simulink library "ammclib_bam_S32K3xx"  (R2016a)
settings: Solver=VariableStepAuto  SolverMode=SingleTasking  StartTime=0.0  StopTime=10.0  RelTol=1e-3
undefined symbols (not defined in the file or in its folder): a1, a2, ADCMaxError, autoCalcEn, b0, b1, b2, cfg, dgain, escale, f16A1, f16A2, f16ADCMaxError, f16B0, f16B1, f16B2, f16C1, f16CC1sc, f16CC1sc_D, f16CC1sc_Q, f16CC2sc, f16CC2sc_D, f16CC2sc_Q, f16DerivGain, f16EGain, f16FiltCoef, f16HystOff, f16HystOn, f16IGain, f16IntegGain, f16IntegGain_D, f16IntegGain_Q, f16IntegGainQ, f16Kd, f16KLs, f16Kq, f16KRs, f16Limit, f16LowerLimit, f16LowerLimit_D, f16LowerLimit_Q, f16LowerLimitQ, f16ModIndex, f16OutValOff, f16OutValOn, f16PropGain, f16PropGain_D, f16PropGain_Q, f16PropGainQ, f16RampDown, f16RampUp, f16UGain, f16UpperLimit, f16UpperLimit_D, f16UpperLimit_Q, f16UpperLimitQ, f16WIGain, f32A1, f32A2, f32ADCMaxError ... (+180)
(part 31 of 50)

== system ammclib_bam_S32K3xx/GFLIB/F16 ==
  GFLIB_Acos_F16 : Subsystem  TreatAsAtomicUnit=on  mask(GFLIB_Acos_F16){}
      mask help: Inverse cosine function in 16-bit fixed-point fractional implementation. Refer to the AMMCLIB User's Guide for further details.
      mask init: same as ammclib_bam_S32K3xx/GDFLIB/F16/GDFLIB_FilterFIR_F16
      settings: RTWSystemCode=Inline
      mask Help: web([fileparts(which('ammclib_bam_S32K3xx.slx')) '/../doc/S32K3XXMCLUG.pdf'], '-browser')
      mask Display: pos = get_param(gcb, 'Position');width = pos(3) - pos(1); height = pos(4) - pos(2);tX=width/2;tY=height - 8;color('black');text(tX,tY, 'GFLIB_Acos_F16', 'horizontalAlignment', 'center');
  GFLIB_Asin_F16 : Subsystem  TreatAsAtomicUnit=on  mask(GFLIB_Asin_F16){}
      mask help: Inverse sine function in 16-bit fixed-point fractional implementation. Refer to the AMMCLIB User's Guide for further details.
      mask init: same as ammclib_bam_S32K3xx/GDFLIB/F16/GDFLIB_FilterFIR_F16
      settings: RTWSystemCode=Inline
      mask Help: web([fileparts(which('ammclib_bam_S32K3xx.slx')) '/../doc/S32K3XXMCLUG.pdf'], '-browser')
      mask Display: pos = get_param(gcb, 'Position');width = pos(3) - pos(1); height = pos(4) - pos(2);tX=width/2;tY=height - 8;color('black');text(tX,tY, 'GFLIB_Asin_F16', 'horizontalAlignment', 'center');
  GFLIB_AtanYXShifted_F16 : Subsystem  TreatAsAtomicUnit=on  mask(GFLIB_AtanYXShifted_F16){}
      mask help: Shifted arctangent of two arguments Y/X in 16-bit fixed-point fractional implementation. Refer to the AMMCLIB User's Guide for further details.
      mask init: same as ammclib_bam_S32K3xx/GDFLIB/F16/GDFLIB_FilterFIR_F16
      settings: RTWSystemCode=Inline
      mask Help: web([fileparts(which('ammclib_bam_S32K3xx.slx')) '/../doc/S32K3XXMCLUG.pdf'], '-browser')
      mask Display: pos = get_param(gcb, 'Position');width = pos(3) - pos(1); height = pos(4) - pos(2);tX=width/2;tY=height - 8;color('black');text(tX,tY, 'GFLIB_AtanYXShifted_F16', 'horizontalAlignment', 'center');
  GFLIB_AtanYX_F16 : Subsystem  TreatAsAtomicUnit=on  mask(GFLIB_AtanYX_F16){}
      mask help: Arctangent of two arguments Y/X in 16-bit fixed-point fractional implementation. Refer to the AMMCLIB User's Guide for further details.
      mask init: same as ammclib_bam_S32K3xx/GDFLIB/F16/GDFLIB_FilterFIR_F16
      settings: RTWSystemCode=Inline
      mask Help: web([fileparts(which('ammclib_bam_S32K3xx.slx')) '/../doc/S32K3XXMCLUG.pdf'], '-browser')
      mask Display: pos = get_param(gcb, 'Position');width = pos(3) - pos(1); height = pos(4) - pos(2);tX=width/2;tY=height - 8;color('black');text(tX,tY, 'GFLIB_AtanYX_F16', 'horizontalAlignment', 'center');
  GFLIB_Atan_F16 : Subsystem  TreatAsAtomicUnit=on  mask(GFLIB_Atan_F16){}
      mask help: Inverse tangent function in 16-bit fixed-point fractional implementation. Refer to the AMMCLIB User's Guide for further details.
      mask init: same as ammclib_bam_S32K3xx/GDFLIB/F16/GDFLIB_FilterFIR_F16
      settings: RTWSystemCode=Inline
      mask Help: web([fileparts(which('ammclib_bam_S32K3xx.slx')) '/../doc/S32K3XXMCLUG.pdf'], '-browser')
      mask Display: pos = get_param(gcb, 'Position');width = pos(3) - pos(1); height = pos(4) - pos(2);tX=width/2;tY=height - 8;color('black');text(tX,tY, 'GFLIB_Atan_F16', 'horizontalAlignment', 'center');
  GFLIB_ControllerPIDpAW_F16 : Subsystem  StartFcn=|  TreatAsAtomicUnit=on  mask(GFLIB_ControllerPIDpAW_F16){showStates=Hide (faster execution), resetStatesEnable=Pre-set according to the first set of inputs after reset, SampleTime=-1, pgain=5, igain=0.5, dgain=0.01, filtCoef=10, lowerLimit=-10, upperLimit=9.99969482421875, inscale=10, outscale=10, autoCalcEn=on, f16PropGain=0, f16IntegGain=0, f16DerivGain=0, f16FiltCoef=0, s16PropGainShift=0, s16IntegGainShift=0, s16DerivGainShift=0, f16LowerLimit=0, f16UpperLimit=0, SampleTime_1=NaN}
      | ts=get_param(gcb,'CompiledSampleTime');
      | if iscell(ts)
      |   ts=ts{1};
      |   if iscell(ts)
      |     ts=ts{1};
      |   end
      | end
      | ts=ts(1);
      | set_param(gcb,'SampleTime_1',num2str(ts));
      | p=Simulink.Mask.get(gcb);
      | hintText=p.getDialogControl('timeHint');
      | SampleTime=Simulink.data.evalinGlobal(bdroot,get_param(gcb,'SampleTime'));
      | p=Simulink.Mask.get(gcb);
      | autoCalcEn=get_param(gcb,'autoCalcEn');
      | if strcmp(autoCalcEn,'on')
      |   if SampleTime==-1
      |     hintText.Prompt='Caution: Implementation parameters depend on inherited sample time. Make sure that the sample time of the block''s inputs corresponds to the sampling period in the target application.';
      |   else
      |     hintText.Prompt='Caution: Implementation parameters depend on the sample time. Make sure that the simulation time step corresponds to the sampling period in the target application.';
      |   end
      |   SampleTime=ts;
      |   f16PropGain_bkup=get_param(gcb,'f16PropGain');
      |   f16IntegGain_bkup=get_param(gcb,'f16IntegGain');
      |   f16DerivGain_bkup=get_param(gcb,'f16DerivGain');
      |   f16FiltCoef_bkup=get_param(gcb,'f16FiltCoef');
      |   s16PropGainShift_bkup=get_param(gcb,'s16PropGainShift');
      |   s16IntegGainShift_bkup=get_param(gcb,'s16IntegGainShift');
      |   s16DerivGainShift_bkup=get_param(gcb,'s16DerivGainShift');
      |   f16LowerLimit_bkup=get_param(gcb,'f16LowerLimit');
      |   f16UpperLimit_bkup=get_param(gcb,'f16UpperLimit');
      |   pgain=Simulink.data.evalinGlobal(bdroot,get_param(gcb,'pgain'));
      |   igain=Simulink.data.evalinGlobal(bdroot,get_param(gcb,'igain'));
      |   dgain=Simulink.data.evalinGlobal(bdroot,get_param(gcb,'dgain'));
      |   filtCoef=Simulink.data.evalinGlobal(bdroot,get_param(gcb,'filtCoef'));
      |   lowerLimit=Simulink.data.evalinGlobal(bdroot,get_param(gcb,'lowerLimit'));
      |   upperLimit=Simulink.data.evalinGlobal(bdroot,get_param(gcb,'upperLimit'));
      |   inscale=Simulink.data.evalinGlobal(bdroot,get_param(gcb,'inscale'));
      |   outscale=Simulink.data.evalinGlobal(bdroot,get_param(gcb,'outscale'));
      |   if (upperLimit<=lowerLimit)
      |     warning('UpperLimit should be greater than LowerLimit.');
      |   end
      |   if (inscale<=0)
      |     warning('E_max must be positive.');
      |   end
      |   if (outscale<=0)
      |     warning('U_max must be positive.');
      |   end
      |   kpf=pgain*inscale/outscale;
      |   s16PropGainShift=ceil(log2(abs(kpf)));
      |   if s16PropGainShift<-15
      |     s16PropGainShift=-15;
      |   end
      |   if s16PropGainShift>15
      |     s16PropGainShift=15;
      |     warning(['Parameter s16PropGainShift of ' gcb ' exceeds the fixed-point range.']);
      |   end
      |   f16PropGain=round(kpf*2^(-s16PropGainShift)*2^15);
      |   if f16PropGain>2^15-1
      |     f16PropGain=2^15-1;
      |     warning(['Parameter f16PropGain of ' gcb ' exceeds the fixed-point range.']);
      |   end
      |   if f16PropGain<-2^15
      |     f16PropGain=-2^15;
      |     warning(['Parameter f16PropGain of ' gcb ' exceeds the fixed-point range.']);
      |   end
      |   kif=igain*SampleTime*0.5*inscale/outscale;
      |   s16IntegGainShift=ceil(log2(abs(kif)));
      |   if s16IntegGainShift<-15
      |     s16IntegGainShift=-15;
      |   end
      |   if s16IntegGainShift>15
      |     s16IntegGainShift=15;
      |     warning(['Parameter s16IntegGainShift of ' gcb ' exceeds the fixed-point range.']);
      |   end
      |   f16IntegGain=round(kif*2^(-s16IntegGainShift)*2^15);
      |   if f16IntegGain>2^15-1
      |     f16IntegGain=2^15-1;
      |     warning(['Parameter f16IntegGain of ' gcb ' exceeds the fixed-point range.']);
      |   end
      |   if f16IntegGain<-2^15
      |     f16IntegGain=-2^15;
      |     warning(['Parameter f16IntegGain of ' gcb ' exceeds the fixed-point range.']);
      |   end
      |   upperLimitf=upperLimit/outscale;
      |   lowerLimitf=lowerLimit/outscale;
      |   f16UpperLimit=round(upperLimitf*2^15);
      |   if f16UpperLimit>2^15-1
      |     f16UpperLimit=2^15-1;
      |     warning(['Parameter f16UpperLimit of ' gcb ' exceeds the fixed-point range.']);
      |   end
      |   if f16UpperLimit<-2^15
      |     f16UpperLimit=-2^15;
      |     warning(['Parameter f16UpperLimit of ' gcb ' exceeds the fixed-point range.']);
      |   end
      |   f16LowerLimit=round(lowerLimitf*2^15);
      |   if f16LowerLimit>2^15-1
      |     f16LowerLimit=2^15-1;
      |     warning(['Parameter f16LowerLimit of ' gcb ' exceeds the fixed-point range.']);
      |   end
      |   if f16LowerLimit<-2^15
      |     f16LowerLimit=-2^15;
      |     warning(['Parameter f16LowerLimit of ' gcb ' exceeds the fixed-point range.']);
      |   end
      |   exparg=-SampleTime*filtCoef;
      |   expconst=exp(exparg);
      |   f16FiltCoef=round(expconst*2^15);
      |   if f16FiltCoef>2^15-1
      |     f16FiltCoef=2^15-1;
      |     warning(['Parameter f16FiltCoef of ' gcb ' exceeds the fixed-point range.']);
      |   end
      |   if f16FiltCoef<-2^15
      |     f16FiltCoef=-2^15;
      |     warning(['Parameter f16FiltCoef of ' gcb ' exceeds the fixed-point range.']);
      |   end
      |   kdf=dgain/SampleTime*(1 - expconst)*inscale/outscale;
      |   s16DerivGainShift=ceil(log2(abs(kpf)));
      |   if s16DerivGainShift<-15
      |     s16DerivGainShift=-15;
      |   end
      |   if s16DerivGainShift>15
      |     s16DerivGainShift=15;
      |     warning(['Parameter s16DerivGainShift of ' gcb ' exceeds the fixed-point range.']);
      |   end
      |   f16DerivGain=round(kpf*2^(-s16DerivGainShift)*2^15);
      |   if f16DerivGain>2^15-1
      |     f16DerivGain=2^15-1;
      |     warning(['Parameter f16DerivGain of ' gcb ' exceeds the fixed-point range.']);
      |   end
      |   if f16DerivGain<-2^15
      |     f16DerivGain=-2^15;
      |     warning(['Parameter f16DerivGain of ' gcb ' exceeds the fixed-point range.']);
      |   end
      |   if isnan(f16PropGain)
      |     if ~strcmp(f16PropGain_bkup,'0')
      |       set_param(gcb,'f16PropGain','0');
      |     end
      |   else
      |     tmps=num2str(f16PropGain);
      |     if ~strcmp(f16PropGain_bkup,tmps)
      |       set_param(gcb,'f16PropGain',tmps);
      |     end
      |   end
      |   if isnan(f16IntegGain)
      |     if ~strcmp(f16IntegGain_bkup,'0')
      |       set_param(gcb,'f16IntegGain','0');
      |     end
      |   else
      |     tmps=num2str(f16IntegGain);
      |     if ~strcmp(f16IntegGain_bkup,tmps)
      |       set_param(gcb,'f16IntegGain',tmps);
      |     end
      |   end
      |   if isnan(f16DerivGain)
      |     if ~strcmp(f16DerivGain_bkup,'0')
      |       set_param(gcb,'f16DerivGain','0');
      |     end
      |   else
      |     tmps=num2str(f16DerivGain);
      |     if ~strcmp(f16DerivGain_bkup,tmps)
      |       set_param(gcb,'f16DerivGain',tmps);
      |     end
      |   end
      |   if isnan(f16FiltCoef)
      |     if ~strcmp(f16FiltCoef_bkup,'0')
      |       set_param(gcb,'f16FiltCoef','0');
      |     end
      |   else
      |     tmps=num2str(f16FiltCoef);
      |     if ~strcmp(f16FiltCoef_bkup,tmps)
      |       set_param(gcb,'f16FiltCoef',tmps);
      |     end
      |   end
      |   if isnan(s16PropGainShift)
      |     if ~strcmp(s16PropGainShift_bkup,'0')
      |       set_param(gcb,'s16PropGainShift','0');
      |     end
      |   else
      |     tmps=num2str(s16PropGainShift);
      |     if ~strcmp(s16PropGainShift_bkup,tmps)
      |       set_param(gcb,'s16PropGainShift',tmps);
      |     end
      |   end
      |   if isnan(s16IntegGainShift)
      |     if ~strcmp(s16IntegGainShift_bkup,'0')
      |       set_param(gcb,'s16IntegGainShift','0');
      |     end
      |   else
      |     tmps=num2str(s16IntegGainShift);
      |     if ~strcmp(s16IntegGainShift_bkup,tmps)
      |       set_param(gcb,'s16IntegGainShift',tmps);
      |     end
      |   end
      |   if isnan(s16DerivGainShift)
      |     if ~strcmp(s16DerivGainShift_bkup,'0')
      |       set_param(gcb,'s16DerivGainShift','0');
      |     end
      |   else
      |     tmps=num2str(s16DerivGainShift);
      |     if ~strcmp(s16DerivGainShift_bkup,tmps)
      |       set_param(gcb,'s16DerivGainShift',tmps);
      |     end
      |   end
      |   if isnan(f16LowerLimit)
      |     if ~strcmp(f16LowerLimit_bkup,'0')
      |       set_param(gcb,'f16LowerLimit','0');
      |     end
      |   else
      |     tmps=num2str(f16LowerLimit);
      |     if ~strcmp(f16LowerLimit_bkup,tmps)
      |       set_param(gcb,'f16LowerLimit',tmps);
      |     end
      |   end
      |   if isnan(f16UpperLimit)
      |     if ~strcmp(f16UpperLimit_bkup,'0')
      |       set_param(gcb,'f16UpperLimit','0');
      |     end
      |   else
      |     tmps=num2str(f16UpperLimit);
      |     if ~strcmp(f16UpperLimit_bkup,tmps)
      |       set_param(gcb,'f16UpperLimit',tmps);
      |     end
      |   end
      | end
      mask prompts: showStates "Show internal states:"; resetStatesEnable "Internal state after reset:"; SampleTime "Sample time (-1 for inherited):"; pgain "Proportional gain (P):"; igain "Integral gain (I):"; dgain "Derivative gain (D):"; filtCoef "Derivative gain limit N (usually 3 to 20):"; lowerLimit "Controller lower limit:"; upperLimit "Controller upper limit:"; inscale "E_max (input scale):"; outscale "U_max (output scale):"; autoCalcEn "Calculate implementation parameters from physical parameters"; f16PropGain "f16PropGain (Proportional gain):"; f16IntegGain "f16IntegGain (Integral gain):"; f16DerivGain "f16DerivGain (Derivative gain):"; f16FiltCoef "f16FiltCoef (Derivative term filter coefficient):"; s16PropGainShift "s16PropGainShift (Proportional gain shift):"; s16IntegGainShift "s16IntegGainShift (Integral gain shift):"; s16DerivGainShift "s16DerivGainShift (Derivative gain shift):"; f16LowerLimit "f16LowerLimit (Lower limit of the controller):"; f16UpperLimit "f16UpperLimit (Upper limit of the controller):"; SampleTime_1 "Discrete sample time:"
      mask help: Parallel form of a discrete-time PID controller with anti-windup in 16-bit fixed-point fractional implementation. This block supports re-initialization of the internal state during simulation. If the block is reset, the controller's output will be aligned with the input f16ControllerPIDpAWOut_preset. Refer to the AMMCLIB User's Guide for further details.
      mask init:
      | ddName = get_param(bdroot,'DataDictionary');
      | if length(ddName)==0
      |   set_param(bdroot,'DataDictionary','ammclib_types.sldd');
      | else
      |   dd = Simulink.data.dictionary.open(ddName);
      |   data = getSection(dd,'Design Data');
      |   if ~exist(data,'SWLIBS_2Syst_F16')
      |     addDataSource(dd,'ammclib_types.sldd');
      |     saveChanges(dd);
      |   end
      | end
      | 
      | if showStates == 1
      |   % hidden state variables
      |   if strcmp(get_param([gcb '/f16PropGain'], 'BlockType'), 'Inport')
      |     posblk = get_param(gcb, 'Position');
      | 
      |     pos = get_param([gcb, '/f16PropGain'], 'Position');
      |     orient = get_param([gcb, '/f16PropGain'], 'Orientation');
      |     delete_block([gcb, '/f16PropGain']);
      |     add_block('built-in/Ground', [gcb, '/f16PropGain'], 'Position', pos, 'Orientation', orient);
      | 
      |     pos = get_param([gcb, '/f16IntegGain'], 'Position');
      |     orient = get_param([gcb, '/f16IntegGain'], 'Orientation');
      |     delete_block([gcb, '/f16IntegGain']);
      |     add_block('built-in/Ground', [gcb, '/f16IntegGain'], 'Position', pos, 'Orientation', orient);
      | 
      |     pos = get_param([gcb, '/f16DerivGain'], 'Position');
      |     orient = get_param([gcb, '/f16DerivGain'], 'Orientation');
      |     delete_block([gcb, '/f16DerivGain']);
      |     add_block('built-in/Ground', [gcb, '/f16DerivGain'], 'Position', pos, 'Orientation', orient);
      | 
      |     pos = get_param([gcb, '/f16FiltCoef'], 'Position');
      |     orient = get_param([gcb, '/f16FiltCoef'], 'Orientation');
      |     delete_block([gcb, '/f16FiltCoef']);
      |     add_block('built-in/Ground', [gcb, '/f16FiltCoef'], 'Position', pos, 'Orientation', orient);
      | 
      |     pos = get_param([gcb, '/s16PropGainShift'], 'Position');
      |     orient = get_param([gcb, '/s16PropGainShift'], 'Orientation');
      |     delete_block([gcb, '/s16PropGainShift']);
      |     add_block('built-in/Ground', [gcb, '/s16PropGainShift'], 'Position', pos, 'Orientation', orient);
      | 
      |     pos = get_param([gcb, '/s16IntegGainShift'], 'Position');
      |     orient = get_param([gcb, '/s16IntegGainShift'], 'Orientation');
      |     delete_block([gcb, '/s16IntegGainShift']);
      |     add_block('built-in/Ground', [gcb, '/s16IntegGainShift'], 'Position', pos, 'Orientation', orient);
      | 
      |     pos = get_param([gcb, '/s16DerivGainShift'], 'Position');
      |     orient = get_param([gcb, '/s16DerivGainShift'], 'Orientation');
      |     delete_block([gcb, '/s16DerivGainShift']);
      |     add_block('built-in/Ground', [gcb, '/s16DerivGainShift'], 'Position', pos, 'Orientation', orient);
      | 
      |     pos = get_param([gcb, '/f16LowerLimit'], 'Position');
      |     orient = get_param([gcb, '/f16LowerLimit'], 'Orientation');
      |     delete_block([gcb, '/f16LowerLimit']);
      |     add_block('built-in/Ground', [gcb, '/f16LowerLimit'], 'Position', pos, 'Orientation', orient);
      | 
      |     pos = get_param([gcb, '/f16UpperLimit'], 'Position');
      |     orient = get_param([gcb, '/f16UpperLimit'], 'Orientation');
      |     delete_block([gcb, '/f16UpperLimit']);
      |     add_block('built-in/Ground', [gcb, '/f16UpperLimit'], 'Position', pos, 'Orientation', orient);
      | 
      |     pos = get_param([gcb, '/f32IntegPartK_1'], 'Position');
      |     orient = get_param([gcb, '/f32IntegPartK_1'], 'Orientation');
      |     delete_block([gcb, '/f32IntegPartK_1']);
      |     add_block('built-in/Ground', [gcb, '/f32IntegPartK_1'], 'Position', pos, 'Orientation', orient);
      | 
      |     pos = get_param([gcb, '/f16DerivPartK_1'], 'Position');
      |     orient = get_param([gcb, '/f16DerivPartK_1'], 'Orientation');
      |     delete_block([gcb, '/f16DerivPartK_1']);
      |     add_block('built-in/Ground', [gcb, '/f16DerivPartK_1'], 'Position', pos, 'Orientation', orient);
      | 
      |     pos = get_param([gcb, '/f16InK_1'], 'Position');
      |     orient = get_param([gcb, '/f16InK_1'], 'Orientation');
      |     delete_block([gcb, '/f16InK_1']);
      |     add_block('built-in/Ground', [gcb, '/f16InK_1'], 'Position', pos, 'Orientation', orient);
      | 
      | 
      |     pmask=Simulink.Mask.get(gcb);
      |     pctrl=pmask.getParameter('SampleTime');
      |     pctrl.set('TypeOptions',{'f16InErr/SampleTime','f16ControllerPIDpAWOut_preset/SampleTime'});
      | 
      |     pos = get_param([gcb '/f32IntegPartK_1_Out'], 'Position');
      |     orient = get_param([gcb '/f32IntegPartK_1_Out'], 'Orientation');
      |     delete_block([gcb '/f32IntegPartK_1_Out']);
      |     add_block('built-in/Terminator', [gcb '/f32IntegPartK_1_Out'], 'Position', pos, 'Orientation', orient);
      | 
      |     pos = get_param([gcb '/f16DerivPartK_1_Out'], 'Position');
      |     orient = get_param([gcb '/f16DerivPartK_1_Out'], 'Orientation');
      |     delete_block([gcb '/f16DerivPartK_1_Out']);
      |     add_block('built-in/Terminator', [gcb '/f16DerivPartK_1_Out'], 'Position', pos, 'Orientation', orient);
      | 
      |     pos = get_param([gcb '/f16InK_1_Out'], 'Position');
      |     orient = get_param([gcb '/f16InK_1_Out'], 'Orientation');
      |     delete_block([gcb '/f16InK_1_Out']);
      |     add_block('built-in/Terminator', [gcb '/f16InK_1_Out'], 'Position', pos, 'Orientation', orient);
      | 
      |     set_param([gcb '/f16InErr'], 'Port', '1');
      |     set_param([gcb '/f16ControllerPIDpAWOut_preset'], 'Port', '2');
      | 
      |     tmpOutCnt=0;
      |     tmpOutCnt=tmpOutCnt+1;
      |     set_param([gcb '/f16Out'], 'Port', num2str(tmpOutCnt));
      |     tmpOutCnt=tmpOutCnt+1;
      |     set_param([gcb '/u16LimitFlag'], 'Port', num2str(tmpOutCnt));
      | 
      |     autoCalcEn=get_param(gcb,'autoCalcEn');
      |     if strcmp(autoCalcEn,'on')
      |       set_param(gcb,'MaskEnables',{'on','on','on','on','on','on','on','on','on','on','on','on','on','on','on','on','on','on','on','on','on','off'});
      |     else
      |       set_param(gcb,'MaskEnables',{'on','on','on','off','off','off','off','off','off','off','off','on','on','on','on','on','on','on','on','on','on','off'});
      |     end
      | 
      |     if (posblk(4) - posblk(2)) > 75
      |       height = 75;
      |       set_param(gcb,'Position',[posblk(1), posblk(2), posblk(3), posblk(2)+height])
      |     end
      |   end
      | else
      |   % shown state variables
      |   if strcmp(get_param([gcb '/f16PropGain'], 'BlockType'), 'Ground')
      |     posblk = get_param(gcb, 'Position');
      | 
      |     pos = get_param([gcb, '/f16PropGain'], 'Position');
      |     orient = get_param([gcb, '/f16PropGain'], 'Orientation');
      |     delete_block([gcb, '/f16PropGain']);
      |     add_block('built-in/Inport', [gcb, '/f16PropGain'], 'Position', pos, 'Orientation', orient, 'OutDataTypeStr', 'int16');
      | 
      |     pos = get_param([gcb, '/f16IntegGain'], 'Position');
      |     orient = get_param([gcb, '/f16IntegGain'], 'Orientation');
      |     delete_block([gcb, '/f16IntegGain']);
      |     add_block('built-in/Inport', [gcb, '/f16IntegGain'], 'Position', pos, 'Orientation', orient, 'OutDataTypeStr', 'int16');
      | 
      |     pos = get_param([gcb, '/f16DerivGain'], 'Position');
      |     orient = get_param([gcb, '/f16DerivGain'], 'Orientation');
      |     delete_block([gcb, '/f16DerivGain']);
      |     add_block('built-in/Inport', [gcb, '/f16DerivGain'], 'Position', pos, 'Orientation', orient, 'OutDataTypeStr', 'int16');
      | 
      |     pos = get_param([gcb, '/f16FiltCoef'], 'Position');
      |     orient = get_param([gcb, '/f16FiltCoef'], 'Orientation');
      |     delete_block([gcb, '/f16FiltCoef']);
      |     add_block('built-in/Inport', [gcb, '/f16FiltCoef'], 'Position', pos, 'Orientation', orient, 'OutDataTypeStr', 'int16');
      | 
      |     pos = get_param([gcb, '/s16PropGainShift'], 'Position');
      |     orient = get_param([gcb, '/s16PropGainShift'], 'Orientation');
      |     delete_block([gcb, '/s16PropGainShift']);
      |     add_block('built-in/Inport', [gcb, '/s16PropGainShift'], 'Position', pos, 'Orientation', orient, 'OutDataTypeStr', 'int16');
      | 
      |     pos = get_param([gcb, '/s16IntegGainShift'], 'Position');
      |     orient = get_param([gcb, '/s16IntegGainShift'], 'Orientation');
      |     delete_block([gcb, '/s16IntegGainShift']);
      |     add_block('built-in/Inport', [gcb, '/s16IntegGainShift'], 'Position', pos, 'Orientation', orient, 'OutDataTypeStr', 'int16');
      | 
      |     pos = get_param([gcb, '/s16DerivGainShift'], 'Position');
      |     orient = get_param([gcb, '/s16DerivGainShift'], 'Orientation');
      |     delete_block([gcb, '/s16DerivGainShift']);
      |     add_block('built-in/Inport', [gcb, '/s16DerivGainShift'], 'Position', pos, 'Orientation', orient, 'OutDataTypeStr', 'int16');
      | 
      |     pos = get_param([gcb, '/f16LowerLimit'], 'Position');
      |     orient = get_param([gcb, '/f16LowerLimit'], 'Orientation');
      |     delete_block([gcb, '/f16LowerLimit']);
      |     add_block('built-in/Inport', [gcb, '/f16LowerLimit'], 'Position', pos, 'Orientation', orient, 'OutDataTypeStr', 'int16');
      | 
      |     pos = get_param([gcb, '/f16UpperLimit'], 'Position');
      |     orient = get_param([gcb, '/f16UpperLimit'], 'Orientation');
      |     delete_block([gcb, '/f16UpperLimit']);
      |     add_block('built-in/Inport', [gcb, '/f16UpperLimit'], 'Position', pos, 'Orientation', orient, 'OutDataTypeStr', 'int16');
      | 
      |     pos = get_param([gcb, '/f32IntegPartK_1'], 'Position');
      |     orient = get_param([gcb, '/f32IntegPartK_1'], 'Orientation');
      |     delete_block([gcb, '/f32IntegPartK_1']);
      |     add_block('built-in/Inport', [gcb, '/f32IntegPartK_1'], 'Position', pos, 'Orientation', orient, 'OutDataTypeStr', 'int32');
      | 
      |     pos = get_param([gcb, '/f16DerivPartK_1'], 'Position');
      |     orient = get_param([gcb, '/f16DerivPartK_1'], 'Orientation');
      |     delete_block([gcb, '/f16DerivPartK_1']);
      |     add_block('built-in/Inport', [gcb, '/f16DerivPartK_1'], 'Position', pos, 'Orientation', orient, 'OutDataTypeStr', 'int16');
      | 
      |     pos = get_param([gcb, '/f16InK_1'], 'Position');
      |     orient = get_param([gcb, '/f16InK_1'], 'Orientation');
      |     delete_block([gcb, '/f16InK_1']);
      |     add_block('built-in/Inport', [gcb, '/f16InK_1'], 'Position', pos, 'Orientation', orient, 'OutDataTypeStr', 'int16');
      | 
      | 
      | 
      |     pos = get_param([gcb '/f32IntegPartK_1_Out'], 'Position');
      |     orient = get_param([gcb '/f32IntegPartK_1_Out'], 'Orientation');
      |     delete_block([gcb '/f32IntegPartK_1_Out']);
      |     add_block('built-in/Outport', [gcb '/f32IntegPartK_1_Out'], 'Position', pos, 'Orientation', orient);
      | 
      |     pos = get_param([gcb '/f16DerivPartK_1_Out'], 'Position');
      |     orient = get_param([gcb '/f16DerivPartK_1_Out'], 'Orientation');
      |     delete_block([gcb '/f16DerivPartK_1_Out']);
      |     add_block('built-in/Outport', [gcb '/f16DerivPartK_1_Out'], 'Position', pos, 'Orientation', orient);
      | 
      |     pos = get_param([gcb '/f16InK_1_Out'], 'Position');
      |     orient = get_param([gcb '/f16InK_1_Out'], 'Orientation');
      |     delete_block([gcb '/f16InK_1_Out']);
      |     add_block('built-in/Outport', [gcb '/f16InK_1_Out'], 'Position', pos, 'Orientation', orient);
      | 
      | 
      |     pmask=Simulink.Mask.get(gcb);
      |     pctrl=pmask.getParameter('SampleTime');
      |     pctrl.set('TypeOptions',{'f16InErr/SampleTime','f16ControllerPIDpAWOut_preset/SampleTime','f16PropGain/SampleTime','f16IntegGain/SampleTime','f16DerivGain/SampleTime','f16FiltCoef/SampleTime','s16PropGainShift/SampleTime','s16IntegGainShift/SampleTime','s16DerivGainShift/SampleTime','f16LowerLimit/SampleTime','f16UpperLimit/SampleTime','f32IntegPartK_1/SampleTime','f16DerivPartK_1/SampleTime','f16InK_1/SampleTime'});
      | 
      |     set_param([gcb '/f16InErr'], 'Port', '1');
      |     set_param([gcb '/f16ControllerPIDpAWOut_preset'], 'Port', '2');
      |     set_param([gcb '/f16PropGain'], 'Port', '3');
      |     set_param([gcb '/f16IntegGain'], 'Port', '4');
      |     set_param([gcb '/f16DerivGain'], 'Port', '5');
      |     set_param([gcb '/f16FiltCoef'], 'Port', '6');
      |     set_param([gcb '/s16PropGainShift'], 'Port', '7');
      |     set_param([gcb '/s16IntegGainShift'], 'Port', '8');
      |     set_param([gcb '/s16DerivGainShift'], 'Port', '9');
      |     set_param([gcb '/f16LowerLimit'], 'Port', '10');
      |     set_param([gcb '/f16UpperLimit'], 'Port', '11');
      |     set_param([gcb '/f32IntegPartK_1'], 'Port', '12');
      |     set_param([gcb '/f16DerivPartK_1'], 'Port', '13');
      |     set_param([gcb '/f16InK_1'], 'Port', '14');
      | 
      |     tmpOutCnt=0;
      |     tmpOutCnt=tmpOutCnt+1;
      |     set_param([gcb '/f16Out'], 'Port', num2str(tmpOutCnt));
      |     tmpOutCnt=tmpOutCnt+1;
      |     set_param([gcb '/u16LimitFlag'], 'Port', num2str(tmpOutCnt));
      |     tmpOutCnt=tmpOutCnt+1;
      |     set_param([gcb '/f32IntegPartK_1_Out'], 'Port', num2str(tmpOutCnt));
      |     tmpOutCnt=tmpOutCnt+1;
      |     set_param([gcb '/f16DerivPartK_1_Out'], 'Port', num2str(tmpOutCnt));
      |     tmpOutCnt=tmpOutCnt+1;
      |     set_param([gcb '/f16InK_1_Out'], 'Port', num2str(tmpOutCnt));
      | 
      |     set_param(gcb,'MaskEnables',{'on','on','on','off','off','off','off','off','off','off','off','off','off','off','off','off','off','off','off','off','off','off'});
      | 
      |     if (posblk(4) - posblk(2)) < 375
      |       height = 375;
      |       set_param(gcb,'Position',[posblk(1), posblk(2), posblk(3), posblk(2)+height])
      |     end
      |   end
      | end
      settings: RTWSystemCode=Inline
      mask Help: web([fileparts(which('ammclib_bam_S32K3xx.slx')) '/../doc/S32K3XXMCLUG.pdf'], '-browser')
      mask TypeOptions showStates: Hide (faster execution) | Show (allows debugging; connect feedback loops manually)
      mask Callback showStates:
      | maskStr=get_param(gcb,'showStates');
      | if strcmp(maskStr,'Hide (faster execution)')
      |   if strcmp(get_param([gcb '/f16PropGain'], 'BlockType'), 'Inport')
      |     autoCalcEn=get_param(gcb,'autoCalcEn');
      |     if strcmp(autoCalcEn,'on')
      |       set_param(gcb,'MaskEnables',{'on','on','on','on','on','on','on','on','on','on','on','on','on','on','on','on','on','on','on','on','on','off'});
      |     else
      |       set_param(gcb,'MaskEnables',{'on','on','on','off','off','off','off','off','off','off','off','on','on','on','on','on','on','on','on','on','on','off'});
      |     end
      |   end
      | else
      |   if strcmp(get_param([gcb '/f16PropGain'], 'BlockType'), 'Ground')
      |     set_param(gcb,'MaskEnables',{'on','on','on','off','off','off','off','off','off','off','off','off','off','off','off','off','off','off','off','off','off','off'});
      |   end
      | end
      mask TypeOptions resetStatesEnable: Pre-set according to the first set of inputs after reset | Clear to zero
      mask TypeOptions SampleTime: f16InErr/SampleTime | f16ControllerPIDpAWOut_preset/SampleTime
      mask Callback SampleTime:
      | p=Simulink.Mask.get(gcb);
      | hintText=p.getDialogControl('timeHint');
      | SampleTime=Simulink.data.evalinGlobal(bdroot,get_param(gcb,'SampleTime'));
      | SampleTime_1=str2double(get_param(gcb,'SampleTime_1'));
      | if (((SampleTime==-1) && (~contains(hintText.Prompt,'inherited'))) || ...
      |     ((SampleTime~=-1) && contains(hintText.Prompt,'inherited')) || ...
      |     ((SampleTime~=-1) && (SampleTime_1~=SampleTime)) || ...
      |     ((SampleTime_1~=-1) && contains(hintText.Prompt,'yet')))
      |   if ((SampleTime==-1) && (~contains(hintText.Prompt,'inherited')))
      |     set_param(gcb,'SampleTime_1',num2str(NaN));
      |     SampleTime_1=NaN;
      |   end
      |   if (SampleTime~=-1)
      |     set_param(gcb,'SampleTime_1',num2str(SampleTime));
      |     SampleTime_1=SampleTime;
      |   end
      |   autoCalcEn=get_param(gcb,'autoCalcEn');
      |   if strcmp(autoCalcEn,'on')
      |     p=Simulink.Mask.get(gcb);
      |     hintText=p.getDialogControl('timeHint');
      |     if SampleTime==-1
      |       SampleTime=SampleTime_1;
      |       if isnan(SampleTime)
      |         hintText.Prompt='Note: Implementation parameters cannot be calculated yet because the block''s inherited sample time is unknown. Simulink will update the sample time when you run the simulation.';
      |       else
      |         hintText.Prompt='Caution: Implementation parameters depend on inherited sample time. Make sure that the sample time of the block''s inputs corresponds to the sampling period in the target application.';
      |       end
      |     else
      |       hintText.Prompt='Caution: Implementation parameters depend on the sample time. Make sure that the simulation time step corresponds to the sampling period in the target application.';
      |     end
      |     f16PropGain_bkup=get_param(gcb,'f16PropGain');
      |     f16IntegGain_bkup=get_param(gcb,'f16IntegGain');
      |     f16DerivGain_bkup=get_param(gcb,'f16DerivGain');
      |     f16FiltCoef_bkup=get_param(gcb,'f16FiltCoef');
      |     s16PropGainShift_bkup=get_param(gcb,'s16PropGainShift');
      |     s16IntegGainShift_bkup=get_param(gcb,'s16IntegGainShift');
      |     s16DerivGainShift_bkup=get_param(gcb,'s16DerivGainShift');
      |     f16LowerLimit_bkup=get_param(gcb,'f16LowerLimit');
      |     f16UpperLimit_bkup=get_param(gcb,'f16UpperLimit');
      |     pgain=Simulink.data.evalinGlobal(bdroot,get_param(gcb,'pgain'));
      |     igain=Simulink.data.evalinGlobal(bdroot,get_param(gcb,'igain'));
      |     dgain=Simulink.data.evalinGlobal(bdroot,get_param(gcb,'dgain'));
      |     filtCoef=Simulink.data.evalinGlobal(bdroot,get_param(gcb,'filtCoef'));
      |     lowerLimit=Simulink.data.evalinGlobal(bdroot,get_param(gcb,'lowerLimit'));
      |     upperLimit=Simulink.data.evalinGlobal(bdroot,get_param(gcb,'upperLimit'));
      |     inscale=Simulink.data.evalinGlobal(bdroot,get_param(gcb,'inscale'));
      |     outscale=Simulink.data.evalinGlobal(bdroot,get_param(gcb,'outscale'));
      |     if (upperLimit<=lowerLimit)
      |       warning('UpperLimit should be greater than LowerLimit.');
      |     end
      |     if (inscale<=0)
      |       warning('E_max must be positive.');
      |     end
      |     if (outscale<=0)
      |       warning('U_max must be positive.');
      |     end
      |     kpf=pgain*inscale/outscale;
      |     s16PropGainShift=ceil(log2(abs(kpf)));
      |     if s16PropGainShift<-15
      |       s16PropGainShift=-15;
      |     end
      |     if s16PropGainShift>15
      |       s16PropGainShift=15;
      |       warning(['Parameter s16PropGainShift of ' gcb ' exceeds the fixed-point range.']);
      |     end
      |     f16PropGain=round(kpf*2^(-s16PropGainShift)*2^15);
      |     if f16PropGain>2^15-1
      |       f16PropGain=2^15-1;
      |       warning(['Parameter f16PropGain of ' gcb ' exceeds the fixed-point range.']);
      |     end
      |     if f16PropGain<-2^15
      |       f16PropGain=-2^15;
      |       warning(['Parameter f16PropGain of ' gcb ' exceeds the fixed-point range.']);
      |     end
      |     kif=igain*SampleTime*0.5*inscale/outscale;
      |     s16IntegGainShift=ceil(log2(abs(kif)));
      |     if s16IntegGainShift<-15
      |       s16IntegGainShift=-15;
      |     end
      |     if s16IntegGainShift>15
      |       s16IntegGainShift=15;
      |       warning(['Parameter s16IntegGainShift of ' gcb ' exceeds the fixed-point range.']);
      |     end
      |     f16IntegGain=round(kif*2^(-s16IntegGainShift)*2^15);
      |     if f16IntegGain>2^15-1
      |       f16IntegGain=2^15-1;
      |       warning(['Parameter f16IntegGain of ' gcb ' exceeds the fixed-point range.']);
      |     end
      |     if f16IntegGain<-2^15
      |       f16IntegGain=-2^15;
      |       warning(['Parameter f16IntegGain of ' gcb ' exceeds the fixed-point range.']);
      |     end
      |     upperLimitf=upperLimit/outscale;
      |     lowerLimitf=lowerLimit/outscale;
      |     f16UpperLimit=round(upperLimitf*2^15);
      |     if f16UpperLimit>2^15-1
      |       f16UpperLimit=2^15-1;
      |       warning(['Parameter f16UpperLimit of ' gcb ' exceeds the fixed-point range.']);
      |     end
      |     if f16UpperLimit<-2^15
      |       f16UpperLimit=-2^15;
      |       warning(['Parameter f16UpperLimit of ' gcb ' exceeds the fixed-point range.']);
      |     end
      |     f16LowerLimit=round(lowerLimitf*2^15);
      |     if f16LowerLimit>2^15-1
      |       f16LowerLimit=2^15-1;
      |       warning(['Parameter f16LowerLimit of ' gcb ' exceeds the fixed-point range.']);
      |     end
      |     if f16LowerLimit<-2^15
      |       f16LowerLimit=-2^15;
      |       warning(['Parameter f16LowerLimit of ' gcb ' exceeds the fixed-point range.']);
      |     end
      |     exparg=-SampleTime*filtCoef;
      |     expconst=exp(exparg);
      |     f16FiltCoef=round(expconst*2^15);
      |     if f16FiltCoef>2^15-1
      |       f16FiltCoef=2^15-1;
      |       warning(['Parameter f16FiltCoef of ' gcb ' exceeds the fixed-point range.']);
      |     end
      |     if f16FiltCoef<-2^15
      |       f16FiltCoef=-2^15;
      |       warning(['Parameter f16FiltCoef of ' gcb ' exceeds the fixed-point range.']);
      |     end
      |     kdf=dgain/SampleTime*(1 - expconst)*inscale/outscale;
      |     s16DerivGainShift=ceil(log2(abs(kpf)));
      |     if s16DerivGainShift<-15
      |       s16DerivGainShift=-15;
      |     end
      |     if s16DerivGainShift>15
      |       s16DerivGainShift=15;
      |       warning(['Parameter s16DerivGainShift of ' gcb ' exceeds the fixed-point range.']);
      |     end
      |     f16DerivGain=round(kpf*2^(-s16DerivGainShift)*2^15);
      |     if f16DerivGain>2^15-1
      |       f16DerivGain=2^15-1;
      |       warning(['Parameter f16DerivGain of ' gcb ' exceeds the fixed-point range.']);
      |     end
      |     if f16DerivGain<-2^15
      |       f16DerivGain=-2^15;
      |       warning(['Parameter f16DerivGain of ' gcb ' exceeds the fixed-point range.']);
      |     end
      |     if isnan(f16PropGain)
      |       if ~strcmp(f16PropGain_bkup,'0')
      |         set_param(gcb,'f16PropGain','0');
      |       end
      |     else
      |       tmps=num2str(f16PropGain);
      |       if ~strcmp(f16PropGain_bkup,tmps)
      |         set_param(gcb,'f16PropGain',tmps);
      |       end
      |     end
      |     if isnan(f16IntegGain)
      |       if ~strcmp(f16IntegGain_bkup,'0')
      |         set_param(gcb,'f16IntegGain','0');
      |       end
      |     else
      |       tmps=num2str(f16IntegGain);
      |       if ~strcmp(f16IntegGain_bkup,tmps)
      |         set_param(gcb,'f16IntegGain',tmps);
      |       end
      |     end
      |     if isnan(f16DerivGain)
      |       if ~strcmp(f16DerivGain_bkup,'0')
      |         set_param(gcb,'f16DerivGain','0');
      |       end
      |     else
      |       tmps=num2str(f16DerivGain);
      |       if ~strcmp(f16DerivGain_bkup,tmps)
      |         set_param(gcb,'f16DerivGain',tmps);
      |       end
      |     end
      |     if isnan(f16FiltCoef)
      |       if ~strcmp(f16FiltCoef_bkup,'0')
      |         set_param(gcb,'f16FiltCoef','0');
      |       end
      |     else
      |       tmps=num2str(f16FiltCoef);
      |       if ~strcmp(f16FiltCoef_bkup,tmps)
      |         set_param(gcb,'f16FiltCoef',tmps);
      |       end
      |     end
      |     if isnan(s16PropGainShift)
      |       if ~strcmp(s16PropGainShift_bkup,'0')
      |         set_param(gcb,'s16PropGainShift','0');
      |       end
      |     else
      |       tmps=num2str(s16PropGainShift);
      |       if ~strcmp(s16PropGainShift_bkup,tmps)
      |         set_param(gcb,'s16PropGainShift',tmps);
      |       end
      |     end
      |     if isnan(s16IntegGainShift)
      |       if ~strcmp(s16IntegGainShift_bkup,'0')
      |         set_param(gcb,'s16IntegGainShift','0');
      |       end
      |     else
      |       tmps=num2str(s16IntegGainShift);
      |       if ~strcmp(s16IntegGainShift_bkup,tmps)
      |         set_param(gcb,'s16IntegGainShift',tmps);
      |       end
      |     end
      |     if isnan(s16DerivGainShift)
      |       if ~strcmp(s16DerivGainShift_bkup,'0')
      |         set_param(gcb,'s16DerivGainShift','0');
      |       end
      |     else
      |       tmps=num2str(s16DerivGainShift);
      |       if ~strcmp(s16DerivGainShift_bkup,tmps)
      |         set_param(gcb,'s16DerivGainShift',tmps);
      |       end
      |     end
      |     if isnan(f16LowerLimit)
      |       if ~strcmp(f16LowerLimit_bkup,'0')
      |         set_param(gcb,'f16LowerLimit','0');
      |       end
      |     else
      |       tmps=num2str(f16LowerLimit);
      |       if ~strcmp(f16LowerLimit_bkup,tmps)
      |         set_param(gcb,'f16LowerLimit',tmps);
      |       end
      |     end
      |     if isnan(f16UpperLimit)
      |       if ~strcmp(f16UpperLimit_bkup,'0')
      |         set_param(gcb,'f16UpperLimit','0');
      |       end
      |     else
      |       tmps=num2str(f16UpperLimit);
      |       if ~strcmp(f16UpperLimit_bkup,tmps)
      |         set_param(gcb,'f16UpperLimit',tmps);
      |       end
      |     end
      |   end
      | end
      mask Callback pgain:
      | autoCalcEn=get_param(gcb,'autoCalcEn');
      | if strcmp(autoCalcEn,'on')
      |   SampleTime=Simulink.data.evalinGlobal(bdroot,get_param(gcb,'SampleTime'));
      |   if (SampleTime==-1)
      |     SampleTime=str2double(get_param(gcb,'SampleTime_1'));
      |   end
      |   f16PropGain_bkup=get_param(gcb,'f16PropGain');
      |   f16IntegGain_bkup=get_param(gcb,'f16IntegGain');
      |   f16DerivGain_bkup=get_param(gcb,'f16DerivGain');
      |   f16FiltCoef_bkup=get_param(gcb,'f16FiltCoef');
      |   s16PropGainShift_bkup=get_param(gcb,'s16PropGainShift');
      |   s16IntegGainShift_bkup=get_param(gcb,'s16IntegGainShift');
      |   s16DerivGainShift_bkup=get_param(gcb,'s16DerivGainShift');
      |   f16LowerLimit_bkup=get_param(gcb,'f16LowerLimit');
      |   f16UpperLimit_bkup=get_param(gcb,'f16UpperLimit');
      |   pgain=Simulink.data.evalinGlobal(bdroot,get_param(gcb,'pgain'));
      |   igain=Simulink.data.evalinGlobal(bdroot,get_param(gcb,'igain'));
      |   dgain=Simulink.data.evalinGlobal(bdroot,get_param(gcb,'dgain'));
      |   filtCoef=Simulink.data.evalinGlobal(bdroot,get_param(gcb,'filtCoef'));
      |   lowerLimit=Simulink.data.evalinGlobal(bdroot,get_param(gcb,'lowerLimit'));
      |   upperLimit=Simulink.data.evalinGlobal(bdroot,get_param(gcb,'upperLimit'));
      |   inscale=Simulink.data.evalinGlobal(bdroot,get_param(gcb,'inscale'));
      |   outscale=Simulink.data.evalinGlobal(bdroot,get_param(gcb,'outscale'));
      |   if (upperLimit<=lowerLimit)
      |     warning('UpperLimit should be greater than LowerLimit.');
      |   end
      |   if (inscale<=0)
      |     warning('E_max must be positive.');
      |   end
      |   if (outscale<=0)
      |     warning('U_max must be positive.');
      |   end
      |   kpf=pgain*inscale/outscale;
      |   s16PropGainShift=ceil(log2(abs(kpf)));
      |   if s16PropGainShift<-15
      |     s16PropGainShift=-15;
      |   end
      |   if s16PropGainShift>15
      |     s16PropGainShift=15;
      |     warning(['Parameter s16PropGainShift of ' gcb ' exceeds the fixed-point range.']);
      |   end
      |   f16PropGain=round(kpf*2^(-s16PropGainShift)*2^15);
      |   if f16PropGain>2^15-1
      |     f16PropGain=2^15-1;
      |     warning(['Parameter f16PropGain of ' gcb ' exceeds the fixed-point range.']);
      |   end
      |   if f16PropGain<-2^15
      |     f16PropGain=-2^15;
      |     warning(['Parameter f16PropGain of ' gcb ' exceeds the fixed-point range.']);
      |   end
      |   kif=igain*SampleTime*0.5*inscale/outscale;
      |   s16IntegGainShift=ceil(log2(abs(kif)));
      |   if s16IntegGainShift<-15
      |     s16IntegGainShift=-15;
      |   end
      |   if s16IntegGainShift>15
      |     s16IntegGainShift=15;
      |     warning(['Parameter s16IntegGainShift of ' gcb ' exceeds the fixed-point range.']);
      |   end
      |   f16IntegGain=round(kif*2^(-s16IntegGainShift)*2^15);
      |   if f16IntegGain>2^15-1
      |     f16IntegGain=2^15-1;
      |     warning(['Parameter f16IntegGain of ' gcb ' exceeds the fixed-point range.']);
      |   end
      |   if f16IntegGain<-2^15
      |     f16IntegGain=-2^15;
      |     warning(['Parameter f16IntegGain of ' gcb ' exceeds the fixed-point range.']);
      |   end
      |   upperLimitf=upperLimit/outscale;
      |   lowerLimitf=lowerLimit/outscale;
      |   f16UpperLimit=round(upperLimitf*2^15);
      |   if f16UpperLimit>2^15-1
      |     f16UpperLimit=2^15-1;
      |     warning(['Parameter f16UpperLimit of ' gcb ' exceeds the fixed-point range.']);
      |   end
      |   if f16UpperLimit<-2^15
      |     f16UpperLimit=-2^15;
      |     warning(['Parameter f16UpperLimit of ' gcb ' exceeds the fixed-point range.']);
      |   end
      |   f16LowerLimit=round(lowerLimitf*2^15);
      |   if f16LowerLimit>2^15-1
      |     f16LowerLimit=2^15-1;
      |     warning(['Parameter f16LowerLimit of ' gcb ' exceeds the fixed-point range.']);
      |   end
      |   if f16LowerLimit<-2^15
      |     f16LowerLimit=-2^15;
      |     warning(['Parameter f16LowerLimit of ' gcb ' exceeds the fixed-point range.']);
      |   end
      |   exparg=-SampleTime*filtCoef;
      |   expconst=exp(exparg);
      |   f16FiltCoef=round(expconst*2^15);
      |   if f16FiltCoef>2^15-1
      |     f16FiltCoef=2^15-1;
      |     warning(['Parameter f16FiltCoef of ' gcb ' exceeds the fixed-point range.']);
      |   end
      |   if f16FiltCoef<-2^15
      |     f16FiltCoef=-2^15;
      |     warning(['Parameter f16FiltCoef of ' gcb ' exceeds the fixed-point range.']);
      |   end
      |   kdf=dgain/SampleTime*(1 - expconst)*inscale/outscale;
      |   s16DerivGainShift=ceil(log2(abs(kpf)));
      |   if s16DerivGainShift<-15
      |     s16DerivGainShift=-15;
      |   end
      |   if s16DerivGainShift>15
      |     s16DerivGainShift=15;
      |     warning(['Parameter s16DerivGainShift of ' gcb ' exceeds the fixed-point range.']);
      |   end
      |   f16DerivGain=round(kpf*2^(-s16DerivGainShift)*2^15);
      |   if f16DerivGain>2^15-1
      |     f16DerivGain=2^15-1;
      |     warning(['Parameter f16DerivGain of ' gcb ' exceeds the fixed-point range.']);
      |   end
      |   if f16DerivGain<-2^15
      |     f16DerivGain=-2^15;
      |     warning(['Parameter f16DerivGain of ' gcb ' exceeds the fixed-point range.']);
      |   end
      |   if isnan(f16PropGain)
      |     if ~strcmp(f16PropGain_bkup,'0')
      |       set_param(gcb,'f16PropGain','0');
      |     end
      |   else
      |     tmps=num2str(f16PropGain);
      |     if ~strcmp(f16PropGain_bkup,tmps)
      |       set_param(gcb,'f16PropGain',tmps);
      |     end
      |   end
      |   if isnan(f16IntegGain)
      |     if ~strcmp(f16IntegGain_bkup,'0')
      |       set_param(gcb,'f16IntegGain','0');
      |     end
      |   else
      |     tmps=num2str(f16IntegGain);
      |     if ~strcmp(f16IntegGain_bkup,tmps)
      |       set_param(gcb,'f16IntegGain',tmps);
      |     end
      |   end
      |   if isnan(f16DerivGain)
      |     if ~strcmp(f16DerivGain_bkup,'0')
      |       set_param(gcb,'f16DerivGain','0');
      |     end
      |   else
      |     tmps=num2str(f16DerivGain);
      |     if ~strcmp(f16DerivGain_bkup,tmps)
      |       set_param(gcb,'f16DerivGain',tmps);
      |     end
      |   end
      |   if isnan(f16FiltCoef)
      |     if ~strcmp(f16FiltCoef_bkup,'0')
      |       set_param(gcb,'f16FiltCoef','0');
      |     end
      |   else
      |     tmps=num2str(f16FiltCoef);
      |     if ~strcmp(f16FiltCoef_bkup,tmps)
      |       set_param(gcb,'f16FiltCoef',tmps);
      |     end
      |   end
      |   if isnan(s16PropGainShift)
      |     if ~strcmp(s16PropGainShift_bkup,'0')
      |       set_param(gcb,'s16PropGainShift','0');
      |     end
      |   else
      |     tmps=num2str(s16PropGainShift);
      |     if ~strcmp(s16PropGainShift_bkup,tmps)
      |       set_param(gcb,'s16PropGainShift',tmps);
      |     end
      |   end
      |   if isnan(s16IntegGainShift)
      |     if ~strcmp(s16IntegGainShift_bkup,'0')
      |       set_param(gcb,'s16IntegGainShift','0');
      |     end
      |   else
      |     tmps=num2str(s16IntegGainShift);
      |     if ~strcmp(s16IntegGainShift_bkup,tmps)
      |       set_param(gcb,'s16IntegGainShift',tmps);
      |     end
      |   end
      |   if isnan(s16DerivGainShift)
      |     if ~strcmp(s16DerivGainShift_bkup,'0')
      |       set_param(gcb,'s16DerivGainShift','0');
      |     end
      |   else
      |     tmps=num2str(s16DerivGainShift);
      |     if ~strcmp(s16DerivGainShift_bkup,tmps)
      |       set_param(gcb,'s16DerivGainShift',tmps);
      |     end
      |   end
      |   if isnan(f16LowerLimit)
      |     if ~strcmp(f16LowerLimit_bkup,'0')
      |       set_param(gcb,'f16LowerLimit','0');
      |     end
      |   else
      |     tmps=num2str(f16LowerLimit);
      |     if ~strcmp(f16LowerLimit_bkup,tmps)
      |       set_param(gcb,'f16LowerLimit',tmps);
      |     end
      |   end
      |   if isnan(f16UpperLimit)
      |     if ~strcmp(f16UpperLimit_bkup,'0')
      |       set_param(gcb,'f16UpperLimit','0');
      |     end
      |   else
      |     tmps=num2str(f16UpperLimit);
      |     if ~strcmp(f16UpperLimit_bkup,tmps)
      |       set_param(gcb,'f16UpperLimit',tmps);
      |     end
      |   end
      | end
      mask Callback igain:
      | autoCalcEn=get_param(gcb,'autoCalcEn');
      | if strcmp(autoCalcEn,'on')
      |   SampleTime=Simulink.data.evalinGlobal(bdroot,get_param(gcb,'SampleTime'));
      |   if (SampleTime==-1)
      |     SampleTime=str2double(get_param(gcb,'SampleTime_1'));
      |   end
      |   f16PropGain_bkup=get_param(gcb,'f16PropGain');
      |   f16IntegGain_bkup=get_param(gcb,'f16IntegGain');
      |   f16DerivGain_bkup=get_param(gcb,'f16DerivGain');
      |   f16FiltCoef_bkup=get_param(gcb,'f16FiltCoef');
      |   s16PropGainShift_bkup=get_param(gcb,'s16PropGainShift');
      |   s16IntegGainShift_bkup=get_param(gcb,'s16IntegGainShift');
      |   s16DerivGainShift_bkup=get_param(gcb,'s16DerivGainShift');
      |   f16LowerLimit_bkup=get_param(gcb,'f16LowerLimit');
      |   f16UpperLimit_bkup=get_param(gcb,'f16UpperLimit');
      |   pgain=Simulink.data.evalinGlobal(bdroot,get_param(gcb,'pgain'));
      |   igain=Simulink.data.evalinGlobal(bdroot,get_param(gcb,'igain'));
      |   dgain=Simulink.data.evalinGlobal(bdroot,get_param(gcb,'dgain'));
      |   filtCoef=Simulink.data.evalinGlobal(bdroot,get_param(gcb,'filtCoef'));
      |   lowerLimit=Simulink.data.evalinGlobal(bdroot,get_param(gcb,'lowerLimit'));
      |   upperLimit=Simulink.data.evalinGlobal(bdroot,get_param(gcb,'upperLimit'));
      |   inscale=Simulink.data.evalinGlobal(bdroot,get_param(gcb,'inscale'));
      |   outscale=Simulink.data.evalinGlobal(bdroot,get_param(gcb,'outscale'));
      |   if (upperLimit<=lowerLimit)
      |     warning('UpperLimit should be greater than LowerLimit.');
      |   end
      |   if (inscale<=0)
      |     warning('E_max must be positive.');
      |   end
      |   if (outscale<=0)
      |     warning('U_max must be positive.');
      |   end
      |   kpf=pgain*inscale/outscale;
      |   s16PropGainShift=ceil(log2(abs(kpf)));
      |   if s16PropGainShift<-15
      |     s16PropGainShift=-15;
      |   end
      |   if s16PropGainShift>15
      |     s16PropGainShift=15;
      |     warning(['Parameter s16PropGainShift of ' gcb ' exceeds the fixed-point range.']);
      |   end
      |   f16PropGain=round(kpf*2^(-s16PropGainShift)*2^15);
      |   if f16PropGain>2^15-1
      |     f16PropGain=2^15-1;
      |     warning(['Parameter f16PropGain of ' gcb ' exceeds the fixed-point range.']);
      |   end
      |   if f16PropGain<-2^15
      |     f16PropGain=-2^15;
      |     warning(['Parameter f16PropGain of ' gcb ' exceeds the fixed-point range.']);
      |   end
      |   kif=igain*SampleTime*0.5*inscale/outscale;
      |   s16IntegGainShift=ceil(log2(abs(kif)));
      |   if s16IntegGainShift<-15
      |     s16IntegGainShift=-15;
      |   end
      |   if s16IntegGainShift>15
      |     s16IntegGainShift=15;
      |     warning(['Parameter s16IntegGainShift of ' gcb ' exceeds the fixed-point range.']);
      |   end
      |   f16IntegGain=round(kif*2^(-s16IntegGainShift)*2^15);
      |   if f16IntegGain>2^15-1
      |     f16IntegGain=2^15-1;
      |     warning(['Parameter f16IntegGain of ' gcb ' exceeds the fixed-point range.']);
      |   end
      |   if f16IntegGain<-2^15
      |     f16IntegGain=-2^15;
      |     warning(['Parameter f16IntegGain of ' gcb ' exceeds the fixed-point range.']);
      |   end
      |   upperLimitf=upperLimit/outscale;
      |   lowerLimitf=lowerLimit/outscale;
      |   f16UpperLimit=round(upperLimitf*2^15);
      |   if f16UpperLimit>2^15-1
      |     f16UpperLimit=2^15-1;
      |     warning(['Parameter f16UpperLimit of ' gcb ' exceeds the fixed-point range.']);
      |   end
      |   if f16UpperLimit<-2^15
      |     f16UpperLimit=-2^15;
      |     warning(['Parameter f16UpperLimit of ' gcb ' exceeds the fixed-point range.']);
      |   end
      |   f16LowerLimit=round(lowerLimitf*2^15);
      |   if f16LowerLimit>2^15-1
      |     f16LowerLimit=2^15-1;
      |     warning(['Parameter f16LowerLimit of ' gcb ' exceeds the fixed-point range.']);
      |   end
      |   if f16LowerLimit<-2^15
      |     f16LowerLimit=-2^15;
      |     warning(['Parameter f16LowerLimit of ' gcb ' exceeds the fixed-point range.']);
      |   end
      |   exparg=-SampleTime*filtCoef;
      |   expconst=exp(exparg);
      |   f16FiltCoef=round(expconst*2^15);
      |   if f16FiltCoef>2^15-1
      |     f16FiltCoef=2^15-1;
      |     warning(['Parameter f16FiltCoef of ' gcb ' exceeds the fixed-point range.']);
      |   end
      |   if f16FiltCoef<-2^15
      |     f16FiltCoef=-2^15;
      |     warning(['Parameter f16FiltCoef of ' gcb ' exceeds the fixed-point range.']);
      |   end
      |   kdf=dgain/SampleTime*(1 - expconst)*inscale/outscale;
      |   s16DerivGainShift=ceil(log2(abs(kpf)));
      |   if s16DerivGainShift<-15
      |     s16DerivGainShift=-15;
      |   end
      |   if s16DerivGainShift>15
      |     s16DerivGainShift=15;
      |     warning(['Parameter s16DerivGainShift of ' gcb ' exceeds the fixed-point range.']);
      |   end
      |   f16DerivGain=round(kpf*2^(-s16DerivGainShift)*2^15);
      |   if f16DerivGain>2^15-1
      |     f16DerivGain=2^15-1;
      |     warning(['Parameter f16DerivGain of ' gcb ' exceeds the fixed-point range.']);
      |   end
      |   if f16DerivGain<-2^15
      |     f16DerivGain=-2^15;
      |     warning(['Parameter f16DerivGain of ' gcb ' exceeds the fixed-point range.']);
      |   end
      |   if isnan(f16PropGain)
      |     if ~strcmp(f16PropGain_bkup,'0')
      |       set_param(gcb,'f16PropGain','0');
      |     end
      |   else
      |     tmps=num2str(f16PropGain);
      |     if ~strcmp(f16PropGain_bkup,tmps)
      |       set_param(gcb,'f16PropGain',tmps);
      |     end
      |   end
      |   if isnan(f16IntegGain)
      |     if ~strcmp(f16IntegGain_bkup,'0')
      |       set_param(gcb,'f16IntegGain','0');
      |     end
      |   else
      |     tmps=num2str(f16IntegGain);
      |     if ~strcmp(f16IntegGain_bkup,tmps)
      |       set_param(gcb,'f16IntegGain',tmps);
      |     end
      |   end
      |   if isnan(f16DerivGain)
      |     if ~strcmp(f16DerivGain_bkup,'0')
      |       set_param(gcb,'f16DerivGain','0');
      |     end
      |   else
      |     tmps=num2str(f16DerivGain);
      |     if ~strcmp(f16DerivGain_bkup,tmps)
      |       set_param(gcb,'f16DerivGain',tmps);
      |     end
      |   end
      |   if isnan(f16FiltCoef)
      |     if ~strcmp(f16FiltCoef_bkup,'0')
      |       set_param(gcb,'f16FiltCoef','0');
      |     end
      |   else
      |     tmps=num2str(f16FiltCoef);
      |     if ~strcmp(f16FiltCoef_bkup,tmps)
      |       set_param(gcb,'f16FiltCoef',tmps);
      |     end
      |   end
      |   if isnan(s16PropGainShift)
      |     if ~strcmp(s16PropGainShift_bkup,'0')
      |       set_param(gcb,'s16PropGainShift','0');
      |     end
      |   else
      |     tmps=num2str(s16PropGainShift);
      |     if ~strcmp(s16PropGainShift_bkup,tmps)
      |       set_param(gcb,'s16PropGainShift',tmps);
      |     end
      |   end
      |   if isnan(s16IntegGainShift)
      |     if ~strcmp(s16IntegGainShift_bkup,'0')
      |       set_param(gcb,'s16IntegGainShift','0');
      |     end
      |   else
      |     tmps=num2str(s16IntegGainShift);
      |     if ~strcmp(s16IntegGainShift_bkup,tmps)
      |       set_param(gcb,'s16IntegGainShift',tmps);
      |     end
      |   end
      |   if isnan(s16DerivGainShift)
      |     if ~strcmp(s16DerivGainShift_bkup,'0')
      |       set_param(gcb,'s16DerivGainShift','0');
      |     end
      |   else
      |     tmps=num2str(s16DerivGainShift);
      |     if ~strcmp(s16DerivGainShift_bkup,tmps)
      |       set_param(gcb,'s16DerivGainShift',tmps);
      |     end
      |   end
      |   if isnan(f16LowerLimit)
      |     if ~strcmp(f16LowerLimit_bkup,'0')
      |       set_param(gcb,'f16LowerLimit','0');
      |     end
      |   else
      |     tmps=num2str(f16LowerLimit);
      |     if ~strcmp(f16LowerLimit_bkup,tmps)
      |       set_param(gcb,'f16LowerLimit',tmps);
      |     end
      |   end
      |   if isnan(f16UpperLimit)
      |     if ~strcmp(f16UpperLimit_bkup,'0')
      |       set_param(gcb,'f16UpperLimit','0');
      |     end
      |   else
      |     tmps=num2str(f16UpperLimit);
      |     if ~strcmp(f16UpperLimit_bkup,tmps)
      |       set_param(gcb,'f16UpperLimit',tmps);
      |     end
      |   end
      | end
      mask Callback dgain:
      | autoCalcEn=get_param(gcb,'autoCalcEn');
      | if strcmp(autoCalcEn,'on')
      |   SampleTime=Simulink.data.evalinGlobal(bdroot,get_param(gcb,'SampleTime'));
      |   if (SampleTime==-1)
      |     SampleTime=str2double(get_param(gcb,'SampleTime_1'));
      |   end
      |   f16PropGain_bkup=get_param(gcb,'f16PropGain');
      |   f16IntegGain_bkup=get_param(gcb,'f16IntegGain');
      |   f16DerivGain_bkup=get_param(gcb,'f16DerivGain');
      |   f16FiltCoef_bkup=get_param(gcb,'f16FiltCoef');
      |   s16PropGainShift_bkup=get_param(gcb,'s16PropGainShift');
      |   s16IntegGainShift_bkup=get_param(gcb,'s16IntegGainShift');
      |   s16DerivGainShift_bkup=get_param(gcb,'s16DerivGainShift');
      |   f16LowerLimit_bkup=get_param(gcb,'f16LowerLimit');
      |   f16UpperLimit_bkup=get_param(gcb,'f16UpperLimit');
      |   pgain=Simulink.data.evalinGlobal(bdroot,get_param(gcb,'pgain'));
      |   igain=Simulink.data.evalinGlobal(bdroot,get_param(gcb,'igain'));
      |   dgain=Simulink.data.evalinGlobal(bdroot,get_param(gcb,'dgain'));
      |   filtCoef=Simulink.data.evalinGlobal(bdroot,get_param(gcb,'filtCoef'));
      |   lowerLimit=Simulink.data.evalinGlobal(bdroot,get_param(gcb,'lowerLimit'));
      |   upperLimit=Simulink.data.evalinGlobal(bdroot,get_param(gcb,'upperLimit'));
      |   inscale=Simulink.data.evalinGlobal(bdroot,get_param(gcb,'inscale'));
      |   outscale=Simulink.data.evalinGlobal(bdroot,get_param(gcb,'outscale'));
      |   if (upperLimit<=lowerLimit)
      |     warning('UpperLimit should be greater than LowerLimit.');
      |   end
      |   if (inscale<=0)
      |     warning('E_max must be positive.');
      |   end
      |   if (outscale<=0)
      |     warning('U_max must be positive.');
      |   end
      |   kpf=pgain*inscale/outscale;
      |   s16PropGainShift=ceil(log2(abs(kpf)));
      |   if s16PropGainShift<-15
      |     s16PropGainShift=-15;
      |   end
      |   if s16PropGainShift>15
      |     s16PropGainShift=15;
      |     warning(['Parameter s16PropGainShift of ' gcb ' exceeds the fixed-point range.']);
      |   end
      |   f16PropGain=round(kpf*2^(-s16PropGainShift)*2^15);
      |   if f16PropGain>2^15-1
      |     f16PropGain=2^15-1;
      |     warning(['Parameter f16PropGain of ' gcb ' exceeds the fixed-point range.']);
      |   end
      |   if f16PropGain<-2^15
      |     f16PropGain=-2^15;
      |     warning(['Parameter f16PropGain of ' gcb ' exceeds the fixed-point range.']);
      |   end
      |   kif=igain*SampleTime*0.5*inscale/outscale;
      |   s16IntegGainShift=ceil(log2(abs(kif)));
      |   if s16IntegGainShift<-15
      |     s16IntegGainShift=-15;
      |   end
      |   if s16IntegGainShift>15
      |     s16IntegGainShift=15;
      |     warning(['Parameter s16IntegGainShift of ' gcb ' exceeds the fixed-point range.']);
      |   end
      |   f16IntegGain=round(kif*2^(-s16IntegGainShift)*2^15);
      |   if f16IntegGain>2^15-1
      |     f16IntegGain=2^15-1;
      |     warning(['Parameter f16IntegGain of ' gcb ' exceeds the fixed-point range.']);
      |   end
      |   if f16IntegGain<-2^15
      |     f16IntegGain=-2^15;
      |     warning(['Parameter f16IntegGain of ' gcb ' exceeds the fixed-point range.']);
      |   end
      |   upperLimitf=upperLimit/outscale;
      |   lowerLimitf=lowerLimit/outscale;
      |   f16UpperLimit=round(upperLimitf*2^15);
      |   if f16UpperLimit>2^15-1
      |     f16UpperLimit=2^15-1;
      |     warning(['Parameter f16UpperLimit of ' gcb ' exceeds the fixed-point range.']);
      |   end
      |   if f16UpperLimit<-2^15
      |     f16UpperLimit=-2^15;
      |     warning(['Parameter f16UpperLimit of ' gcb ' exceeds the fixed-point range.']);
      |   end
      |   f16LowerLimit=round(lowerLimitf*2^15);
      |   if f16LowerLimit>2^15-1
      |     f16LowerLimit=2^15-1;
      |     warning(['Parameter f16LowerLimit of ' gcb ' exceeds the fixed-point range.']);
      |   end
      |   if f16LowerLimit<-2^15
      |     f16LowerLimit=-2^15;
      |     warning(['Parameter f16LowerLimit of ' gcb ' exceeds the fixed-point range.']);
      |   end
      |   exparg=-SampleTime*filtCoef;
      |   expconst=exp(exparg);
      |   f16FiltCoef=round(expconst*2^15);
      |   if f16FiltCoef>2^15-1
      |     f16FiltCoef=2^15-1;
      |     warning(['Parameter f16FiltCoef of ' gcb ' exceeds the fixed-point range.']);
      |   end
      |   if f16FiltCoef<-2^15
      |     f16FiltCoef=-2^15;
      |     warning(['Parameter f16FiltCoef of ' gcb ' exceeds the fixed-point range.']);
      |   end
      |   kdf=dgain/SampleTime*(1 - expconst)*inscale/outscale;
      |   s16DerivGainShift=ceil(log2(abs(kpf)));
      |   if s16DerivGainShift<-15
      |     s16DerivGainShift=-15;
      |   end
      |   if s16DerivGainShift>15
      |     s16DerivGainShift=15;
      |     warning(['Parameter s16DerivGainShift of ' gcb ' exceeds the fixed-point range.']);
      |   end
      |   f16DerivGain=round(kpf*2^(-s16DerivGainShift)*2^15);
      |   if f16DerivGain>2^15-1
      |     f16DerivGain=2^15-1;
      |     warning(['Parameter f16DerivGain of ' gcb ' exceeds the fixed-point range.']);
      |   end
      |   if f16DerivGain<-2^15
      |     f16DerivGain=-2^15;
      |     warning(['Parameter f16DerivGain of ' gcb ' exceeds the fixed-point range.']);
      |   end
      |   if isnan(f16PropGain)
      |     if ~strcmp(f16PropGain_bkup,'0')
      |       set_param(gcb,'f16PropGain','0');
      |     end
      |   else
      |     tmps=num2str(f16PropGain);
      |     if ~strcmp(f16PropGain_bkup,tmps)
      |       set_param(gcb,'f16PropGain',tmps);
      |     end
      |   end
      |   if isnan(f16IntegGain)
      |     if ~strcmp(f16IntegGain_bkup,'0')
      |       set_param(gcb,'f16IntegGain','0');
      |     end
      |   else
      |     tmps=num2str(f16IntegGain);
      |     if ~strcmp(f16IntegGain_bkup,tmps)
      |       set_param(gcb,'f16IntegGain',tmps);
      |     end
      |   end
      |   if isnan(f16DerivGain)
      |     if ~strcmp(f16DerivGain_bkup,'0')
      |       set_param(gcb,'f16DerivGain','0');
      |     end
      |   else
      |     tmps=num2str(f16DerivGain);
      |     if ~strcmp(f16DerivGain_bkup,tmps)
      |       set_param(gcb,'f16DerivGain',tmps);
      |     end
      |   end
      |   if isnan(f16FiltCoef)
      |     if ~strcmp(f16FiltCoef_bkup,'0')
      |       set_param(gcb,'f16FiltCoef','0');
      |     end
      |   else
      |     tmps=num2str(f16FiltCoef);
      |     if ~strcmp(f16FiltCoef_bkup,tmps)
      |       set_param(gcb,'f16FiltCoef',tmps);
      |     end
      |   end
      |   if isnan(s16PropGainShift)
      |     if ~strcmp(s16PropGainShift_bkup,'0')
      |       set_param(gcb,'s16PropGainShift','0');
      |     end
      |   else
      |     tmps=num2str(s16PropGainShift);
      |     if ~strcmp(s16PropGainShift_bkup,tmps)
      |       set_param(gcb,'s16PropGainShift',tmps);
      |     end
      |   end
      |   if isnan(s16IntegGainShift)
      |     if ~strcmp(s16IntegGainShift_bkup,'0')
      |       set_param(gcb,'s16IntegGainShift','0');
      |     end
      |   else
      |     tmps=num2str(s16IntegGainShift);
      |     if ~strcmp(s16IntegGainShift_bkup,tmps)
      |       set_param(gcb,'s16IntegGainShift',tmps);
      |     end
      |   end
      |   if isnan(s16DerivGainShift)
      |     if ~strcmp(s16DerivGainShift_bkup,'0')
      |       set_param(gcb,'s16DerivGainShift','0');
      |     end
      |   else
      |     tmps=num2str(s16DerivGainShift);
      |     if ~strcmp(s16DerivGainShift_bkup,tmps)
      |       set_param(gcb,'s16DerivGainShift',tmps);
      |     end
      |   end
      |   if isnan(f16LowerLimit)
      |     if ~strcmp(f16LowerLimit_bkup,'0')
      |       set_param(gcb,'f16LowerLimit','0');
      |     end
      |   else
      |     tmps=num2str(f16LowerLimit);
      |     if ~strcmp(f16LowerLimit_bkup,tmps)
      |       set_param(gcb,'f16LowerLimit',tmps);
      |     end
      |   end
      |   if isnan(f16UpperLimit)
      |     if ~strcmp(f16UpperLimit_bkup,'0')
      |       set_param(gcb,'f16UpperLimit','0');
      |     end
      |   else
      |     tmps=num2str(f16UpperLimit);
      |     if ~strcmp(f16UpperLimit_bkup,tmps)
      |       set_param(gcb,'f16UpperLimit',tmps);
      |     end
      |   end
      | end
      mask Callback filtCoef:
      | autoCalcEn=get_param(gcb,'autoCalcEn');
      | if strcmp(autoCalcEn,'on')
      |   SampleTime=Simulink.data.evalinGlobal(bdroot,get_param(gcb,'SampleTime'));
      |   if (SampleTime==-1)
      |     SampleTime=str2double(get_param(gcb,'SampleTime_1'));
      |   end
      |   f16PropGain_bkup=get_param(gcb,'f16PropGain');
      |   f16IntegGain_bkup=get_param(gcb,'f16IntegGain');
      |   f16DerivGain_bkup=get_param(gcb,'f16DerivGain');
      |   f16FiltCoef_bkup=get_param(gcb,'f16FiltCoef');
      |   s16PropGainShift_bkup=get_param(gcb,'s16PropGainShift');
      |   s16IntegGainShift_bkup=get_param(gcb,'s16IntegGainShift');
      |   s16DerivGainShift_bkup=get_param(gcb,'s16DerivGainShift');
      |   f16LowerLimit_bkup=get_param(gcb,'f16LowerLimit');
      |   f16UpperLimit_bkup=get_param(gcb,'f16UpperLimit');
      |   pgain=Simulink.data.evalinGlobal(bdroot,get_param(gcb,'pgain'));
      |   igain=Simulink.data.evalinGlobal(bdroot,get_param(gcb,'igain'));
      |   dgain=Simulink.data.evalinGlobal(bdroot,get_param(gcb,'dgain'));
      |   filtCoef=Simulink.data.evalinGlobal(bdroot,get_param(gcb,'filtCoef'));
      |   lowerLimit=Simulink.data.evalinGlobal(bdroot,get_param(gcb,'lowerLimit'));
      |   upperLimit=Simulink.data.evalinGlobal(bdroot,get_param(gcb,'upperLimit'));
      |   inscale=Simulink.data.evalinGlobal(bdroot,get_param(gcb,'inscale'));
      |   outscale=Simulink.data.evalinGlobal(bdroot,get_param(gcb,'outscale'));
      |   if (upperLimit<=lowerLimit)
      |     warning('UpperLimit should be greater than LowerLimit.');
      |   end
      |   if (inscale<=0)
      |     warning('E_max must be positive.');
      |   end
      |   if (outscale<=0)
      |     warning('U_max must be positive.');
      |   end
      |   kpf=pgain*inscale/outscale;
      |   s16PropGainShift=ceil(log2(abs(kpf)));
      |   if s16PropGainShift<-15
      |     s16PropGainShift=-15;
      |   end
      |   if s16PropGainShift>15
      |     s16PropGainShift=15;
      |     warning(['Parameter s16PropGainShift of ' gcb ' exceeds the fixed-point range.']);
      |   end
      |   f16PropGain=round(kpf*2^(-s16PropGainShift)*2^15);
      |   if f16PropGain>2^15-1
      |     f16PropGain=2^15-1;
      |     warning(['Parameter f16PropGain of ' gcb ' exceeds the fixed-point range.']);
      |   end
      |   if f16PropGain<-2^15
      |     f16PropGain=-2^15;
      |     warning(['Parameter f16PropGain of ' gcb ' exceeds the fixed-point range.']);
      |   end
      |   kif=igain*SampleTime*0.5*inscale/outscale;
      |   s16IntegGainShift=ceil(log2(abs(kif)));
      |   if s16IntegGainShift<-15
      |     s16IntegGainShift=-15;
      |   end
      |   if s16IntegGainShift>15
      |     s16IntegGainShift=15;
      |     warning(['Parameter s16IntegGainShift of ' gcb ' exceeds the fixed-point range.']);
      |   end
      |   f16IntegGain=round(kif*2^(-s16IntegGainShift)*2^15);
      |   if f16IntegGain>2^15-1
      |     f16IntegGain=2^15-1;
      |     warning(['Parameter f16IntegGain of ' gcb ' exceeds the fixed-point range.']);
      |   end
      |   if f16IntegGain<-2^15
      |     f16IntegGain=-2^15;
      |     warning(['Parameter f16IntegGain of ' gcb ' exceeds the fixed-point range.']);
      |   end
      |   upperLimitf=upperLimit/outscale;
      |   lowerLimitf=lowerLimit/outscale;
      |   f16UpperLimit=round(upperLimitf*2^15);
      |   if f16UpperLimit>2^15-1
      |     f16UpperLimit=2^15-1;
      |     warning(['Parameter f16UpperLimit of ' gcb ' exceeds the fixed-point range.']);
      |   end
      |   if f16UpperLimit<-2^15
      |     f16UpperLimit=-2^15;
      |     warning(['Parameter f16UpperLimit of ' gcb ' exceeds the fixed-point range.']);
      |   end
      |   f16LowerLimit=round(lowerLimitf*2^15);
      |   if f16LowerLimit>2^15-1
      |     f16LowerLimit=2^15-1;
      |     warning(['Parameter f16LowerLimit of ' gcb ' exceeds the fixed-point range.']);
      |   end
      |   if f16LowerLimit<-2^15
      |     f16LowerLimit=-2^15;
      |     warning(['Parameter f16LowerLimit of ' gcb ' exceeds the fixed-point range.']);
      |   end
      |   exparg=-SampleTime*filtCoef;
      |   expconst=exp(exparg);
      |   f16FiltCoef=round(expconst*2^15);
      |   if f16FiltCoef>2^15-1
      |     f16FiltCoef=2^15-1;
      |     warning(['Parameter f16FiltCoef of ' gcb ' exceeds the fixed-point range.']);
      |   end
      |   if f16FiltCoef<-2^15
      |     f16FiltCoef=-2^15;
      |     warning(['Parameter f16FiltCoef of ' gcb ' exceeds the fixed-point range.']);
      |   end
      |   kdf=dgain/SampleTime*(1 - expconst)*inscale/outscale;
      |   s16DerivGainShift=ceil(log2(abs(kpf)));
      |   if s16DerivGainShift<-15
      |     s16DerivGainShift=-15;
      |   end
      |   if s16DerivGainShift>15
      |     s16DerivGainShift=15;
      |     warning(['Parameter s16DerivGainShift of ' gcb ' exceeds the fixed-point range.']);
      |   end
      |   f16DerivGain=round(kpf*2^(-s16DerivGainShift)*2^15);
      |   if f16DerivGain>2^15-1
      |     f16DerivGain=2^15-1;
      |     warning(['Parameter f16DerivGain of ' gcb ' exceeds the fixed-point range.']);
      |   end
      |   if f16DerivGain<-2^15
      |     f16DerivGain=-2^15;
      |     warning(['Parameter f16DerivGain of ' gcb ' exceeds the fixed-point range.']);
      |   end
      |   if isnan(f16PropGain)
      |     if ~strcmp(f16PropGain_bkup,'0')
      |       set_param(gcb,'f16PropGain','0');
      |     end
      |   else
      |     tmps=num2str(f16PropGain);
      |     if ~strcmp(f16PropGain_bkup,tmps)
      |       set_param(gcb,'f16PropGain',tmps);
      |     end
      |   end
      |   if isnan(f16IntegGain)
      |     if ~strcmp(f16IntegGain_bkup,'0')
      |       set_param(gcb,'f16IntegGain','0');
      |     end
      |   else
      |     tmps=num2str(f16IntegGain);
      |     if ~strcmp(f16IntegGain_bkup,tmps)
      |       set_param(gcb,'f16IntegGain',tmps);
      |     end
      |   end
      |   if isnan(f16DerivGain)
      |     if ~strcmp(f16DerivGain_bkup,'0')
      |       set_param(gcb,'f16DerivGain','0');
      |     end
      |   else
      |     tmps=num2str(f16DerivGain);
      |     if ~strcmp(f16DerivGain_bkup,tmps)
      |       set_param(gcb,'f16DerivGain',tmps);
      |     end
      |   end
      |   if isnan(f16FiltCoef)
      |     if ~strcmp(f16FiltCoef_bkup,'0')
      |       set_param(gcb,'f16FiltCoef','0');
      |     end
      |   else
      |     tmps=num2str(f16FiltCoef);
      |     if ~strcmp(f16FiltCoef_bkup,tmps)
      |       set_param(gcb,'f16FiltCoef',tmps);
      |     end
      |   end
      |   if isnan(s16PropGainShift)
      |     if ~strcmp(s16PropGainShift_bkup,'0')
      |       set_param(gcb,'s16PropGainShift','0');
      |     end
      |   else
      |     tmps=num2str(s16PropGainShift);
      |     if ~strcmp(s16PropGainShift_bkup,tmps)
      |       set_param(gcb,'s16PropGainShift',tmps);
      |     end
      |   end
      |   if isnan(s16IntegGainShift)
      |     if ~strcmp(s16IntegGainShift_bkup,'0')
      |       set_param(gcb,'s16IntegGainShift','0');
      |     end
      |   else
      |     tmps=num2str(s16IntegGainShift);
      |     if ~strcmp(s16IntegGainShift_bkup,tmps)
      |       set_param(gcb,'s16IntegGainShift',tmps);
      |     end
      |   end
      |   if isnan(s16DerivGainShift)
      |     if ~strcmp(s16DerivGainShift_bkup,'0')
      |       set_param(gcb,'s16DerivGainShift','0');
      |     end
      |   else
      |     tmps=num2str(s16DerivGainShift);
      |     if ~strcmp(s16DerivGainShift_bkup,tmps)
      |       set_param(gcb,'s16DerivGainShift',tmps);
      |     end
      |   end
      |   if isnan(f16LowerLimit)
      |     if ~strcmp(f16LowerLimit_bkup,'0')
      |       set_param(gcb,'f16LowerLimit','0');
      |     end
      |   else
      |     tmps=num2str(f16LowerLimit);
      |     if ~strcmp(f16LowerLimit_bkup,tmps)
      |       set_param(gcb,'f16LowerLimit',tmps);
      |     end
      |   end
      |   if isnan(f16UpperLimit)
      |     if ~strcmp(f16UpperLimit_bkup,'0')
      |       set_param(gcb,'f16UpperLimit','0');
      |     end
      |   else
      |     tmps=num2str(f16UpperLimit);
      |     if ~strcmp(f16UpperLimit_bkup,tmps)
      |       set_param(gcb,'f16UpperLimit',tmps);
      |     end
      |   end
      | end
      mask Callback lowerLimit:
      | autoCalcEn=get_param(gcb,'autoCalcEn');
      | if strcmp(autoCalcEn,'on')
      |   SampleTime=Simulink.data.evalinGlobal(bdroot,get_param(gcb,'SampleTime'));
      |   if (SampleTime==-1)
      |     SampleTime=str2double(get_param(gcb,'SampleTime_1'));
      |   end
      |   f16PropGain_bkup=get_param(gcb,'f16PropGain');
      |   f16IntegGain_bkup=get_param(gcb,'f16IntegGain');
      |   f16DerivGain_bkup=get_param(gcb,'f16DerivGain');
      |   f16FiltCoef_bkup=get_param(gcb,'f16FiltCoef');
      |   s16PropGainShift_bkup=get_param(gcb,'s16PropGainShift');
      |   s16IntegGainShift_bkup=get_param(gcb,'s16IntegGainShift');
      |   s16DerivGainShift_bkup=get_param(gcb,'s16DerivGainShift');
      |   f16LowerLimit_bkup=get_param(gcb,'f16LowerLimit');
      |   f16UpperLimit_bkup=get_param(gcb,'f16UpperLimit');
      |   pgain=Simulink.data.evalinGlobal(bdroot,get_param(gcb,'pgain'));
      |   igain=Simulink.data.evalinGlobal(bdroot,get_param(gcb,'igain'));
      |   dgain=Simulink.data.evalinGlobal(bdroot,get_param(gcb,'dgain'));
      |   filtCoef=Simulink.data.evalinGlobal(bdroot,get_param(gcb,'filtCoef'));
      |   lowerLimit=Simulink.data.evalinGlobal(bdroot,get_param(gcb,'lowerLimit'));
      |   upperLimit=Simulink.data.evalinGlobal(bdroot,get_param(gcb,'upperLimit'));
      |   inscale=Simulink.data.evalinGlobal(bdroot,get_param(gcb,'inscale'));
      |   outscale=Simulink.data.evalinGlobal(bdroot,get_param(gcb,'outscale'));
      |   if (upperLimit<=lowerLimit)
      |     warning('UpperLimit should be greater than LowerLimit.');
      |   end
      |   if (inscale<=0)
      |     warning('E_max must be positive.');
      |   end
      |   if (outscale<=0)
      |     warning('U_max must be positive.');
      |   end
      |   kpf=pgain*inscale/outscale;
      |   s16PropGainShift=ceil(log2(abs(kpf)));
      |   if s16PropGainShift<-15
      |     s16PropGainShift=-15;
      |   end
      |   if s16PropGainShift>15
      |     s16PropGainShift=15;
      |     warning(['Parameter s16PropGainShift of ' gcb ' exceeds the fixed-point range.']);
      |   end
      |   f16PropGain=round(kpf*2^(-s16PropGainShift)*2^15);
      |   if f16PropGain>2^15-1
      |     f16PropGain=2^15-1;
      |     warning(['Parameter f16PropGain of ' gcb ' exceeds the fixed-point range.']);
      |   end
      |   if f16PropGain<-2^15
      |     f16PropGain=-2^15;
      |     warning(['Parameter f16PropGain of ' gcb ' exceeds the fixed-point range.']);
      |   end
      |   kif=igain*SampleTime*0.5*inscale/outscale;
      |   s16IntegGainShift=ceil(log2(abs(kif)));
      |   if s16IntegGainShift<-15
      |     s16IntegGainShift=-15;
      |   end
      |   if s16IntegGainShift>15
      |     s16IntegGainShift=15;
      |     warning(['Parameter s16IntegGainShift of ' gcb ' exceeds the fixed-point range.']);
      |   end
      |   f16IntegGain=round(kif*2^(-s16IntegGainShift)*2^15);
      |   if f16IntegGain>2^15-1
      |     f16IntegGain=2^15-1;
      |     warning(['Parameter f16IntegGain of ' gcb ' exceeds the fixed-point range.']);
      |   end
      |   if f16IntegGain<-2^15
      |     f16IntegGain=-2^15;
      |     warning(['Parameter f16IntegGain of ' gcb ' exceeds the fixed-point range.']);
      |   end
      |   upperLimitf=upperLimit/outscale;
      |   lowerLimitf=lowerLimit/outscale;
      |   f16UpperLimit=round(upperLimitf*2^15);
      |   if f16UpperLimit>2^15-1
      |     f16UpperLimit=2^15-1;
      |     warning(['Parameter f16UpperLimit of ' gcb ' exceeds the fixed-point range.']);
      |   end
      |   if f16UpperLimit<-2^15
      |     f16UpperLimit=-2^15;
      |     warning(['Parameter f16UpperLimit of ' gcb ' exceeds the fixed-point range.']);
      |   end
      |   f16LowerLimit=round(lowerLimitf*2^15);
      |   if f16LowerLimit>2^15-1
      |     f16LowerLimit=2^15-1;
      |     warning(['Parameter f16LowerLimit of ' gcb ' exceeds the fixed-point range.']);
      |   end
      |   if f16LowerLimit<-2^15
      |     f16LowerLimit=-2^15;
      |     warning(['Parameter f16LowerLimit of ' gcb ' exceeds the fixed-point range.']);
      |   end
      |   exparg=-SampleTime*filtCoef;
      |   expconst=exp(exparg);
      |   f16FiltCoef=round(expconst*2^15);
      |   if f16FiltCoef>2^15-1
      |     f16FiltCoef=2^15-1;
      |     warning(['Parameter f16FiltCoef of ' gcb ' exceeds the fixed-point range.']);
      |   end
      |   if f16FiltCoef<-2^15
      |     f16FiltCoef=-2^15;
      |     warning(['Parameter f16FiltCoef of ' gcb ' exceeds the fixed-point range.']);
      |   end
      |   kdf=dgain/SampleTime*(1 - expconst)*inscale/outscale;
      |   s16DerivGainShift=ceil(log2(abs(kpf)));
      |   if s16DerivGainShift<-15
      |     s16DerivGainShift=-15;
      |   end
      |   if s16DerivGainShift>15
      |     s16DerivGainShift=15;
      |     warning(['Parameter s16DerivGainShift of ' gcb ' exceeds the fixed-point range.']);
      |   end
      |   f16DerivGain=round(kpf*2^(-s16DerivGainShift)*2^15);
      |   if f16DerivGain>2^15-1
      |     f16DerivGain=2^15-1;
      |     warning(['Parameter f16DerivGain of ' gcb ' exceeds the fixed-point range.']);
      |   end
      |   if f16DerivGain<-2^15
      |     f16DerivGain=-2^15;
      |     warning(['Parameter f16DerivGain of ' gcb ' exceeds the fixed-point range.']);
      |   end
      |   if isnan(f16PropGain)
      |     if ~strcmp(f16PropGain_bkup,'0')
      |       set_param(gcb,'f16PropGain','0');
      |     end
      |   else
      |     tmps=num2str(f16PropGain);
      |     if ~strcmp(f16PropGain_bkup,tmps)
      |       set_param(gcb,'f16PropGain',tmps);
      |     end
      |   end
      |   if isnan(f16IntegGain)
      |     if ~strcmp(f16IntegGain_bkup,'0')
      |       set_param(gcb,'f16IntegGain','0');
      |     end
      |   else
      |     tmps=num2str(f16IntegGain);
      |     if ~strcmp(f16IntegGain_bkup,tmps)
      |       set_param(gcb,'f16IntegGain',tmps);
      |     end
      |   end
      |   if isnan(f16DerivGain)
      |     if ~strcmp(f16DerivGain_bkup,'0')
      |       set_param(gcb,'f16DerivGain','0');
      |     end
      |   else
      |     tmps=num2str(f16DerivGain);
      |     if ~strcmp(f16DerivGain_bkup,tmps)
      |       set_param(gcb,'f16DerivGain',tmps);
      |     end
      |   end
      |   if isnan(f16FiltCoef)
      |     if ~strcmp(f16FiltCoef_bkup,'0')
      |       set_param(gcb,'f16FiltCoef','0');
      |     end
      |   else
      |     tmps=num2str(f16FiltCoef);
      |     if ~strcmp(f16FiltCoef_bkup,tmps)
      |       set_param(gcb,'f16FiltCoef',tmps);
      |     end
      |   end
      |   if isnan(s16PropGainShift)
      |     if ~strcmp(s16PropGainShift_bkup,'0')
      |       set_param(gcb,'s16PropGainShift','0');
      |     end
      |   else
      |     tmps=num2str(s16PropGainShift);
      |     if ~strcmp(s16PropGainShift_bkup,tmps)
      |       set_param(gcb,'s16PropGainShift',tmps);
      |     end
      |   end
      |   if isnan(s16IntegGainShift)
      |     if ~strcmp(s16IntegGainShift_bkup,'0')
      |       set_param(gcb,'s16IntegGainShift','0');
      |     end
      |   else
      |     tmps=num2str(s16IntegGainShift);
      |     if ~strcmp(s16IntegGainShift_bkup,tmps)
      |       set_param(gcb,'s16IntegGainShift',tmps);
      |     end
      |   end
      |   if isnan(s16DerivGainShift)
      |     if ~strcmp(s16DerivGainShift_bkup,'0')
      |       set_param(gcb,'s16DerivGainShift','0');
      |     end
      |   else
      |     tmps=num2str(s16DerivGainShift);
      |     if ~strcmp(s16DerivGainShift_bkup,tmps)
      |       set_param(gcb,'s16DerivGainShift',tmps);
      |     end
      |   end
      |   if isnan(f16LowerLimit)
      |     if ~strcmp(f16LowerLimit_bkup,'0')
      |       set_param(gcb,'f16LowerLimit','0');
      |     end
      |   else
      |     tmps=num2str(f16LowerLimit);
      |     if ~strcmp(f16LowerLimit_bkup,tmps)
      |       set_param(gcb,'f16LowerLimit',tmps);
      |     end
      |   end
      |   if isnan(f16UpperLimit)
      |     if ~strcmp(f16UpperLimit_bkup,'0')
      |       set_param(gcb,'f16UpperLimit','0');
      |     end
      |   else
      |     tmps=num2str(f16UpperLimit);
      |     if ~strcmp(f16UpperLimit_bkup,tmps)
      |       set_param(gcb,'f16UpperLimit',tmps);
      |     end
      |   end
      | end
      mask Callback upperLimit:
      | autoCalcEn=get_param(gcb,'autoCalcEn');
      | if strcmp(autoCalcEn,'on')
      |   SampleTime=Simulink.data.evalinGlobal(bdroot,get_param(gcb,'SampleTime'));
      |   if (SampleTime==-1)
      |     SampleTime=str2double(get_param(gcb,'SampleTime_1'));
      |   end
      |   f16PropGain_bkup=get_param(gcb,'f16PropGain');
      |   f16IntegGain_bkup=get_param(gcb,'f16IntegGain');
      |   f16DerivGain_bkup=get_param(gcb,'f16DerivGain');
      |   f16FiltCoef_bkup=get_param(gcb,'f16FiltCoef');
      |   s16PropGainShift_bkup=get_param(gcb,'s16PropGainShift');
      |   s16IntegGainShift_bkup=get_param(gcb,'s16IntegGainShift');
      |   s16DerivGainShift_bkup=get_param(gcb,'s16DerivGainShift');
      |   f16LowerLimit_bkup=get_param(gcb,'f16LowerLimit');
      |   f16UpperLimit_bkup=get_param(gcb,'f16UpperLimit');
      |   pgain=Simulink.data.evalinGlobal(bdroot,get_param(gcb,'pgain'));
      |   igain=Simulink.data.evalinGlobal(bdroot,get_param(gcb,'igain'));
      |   dgain=Simulink.data.evalinGlobal(bdroot,get_param(gcb,'dgain'));
      |   filtCoef=Simulink.data.evalinGlobal(bdroot,get_param(gcb,'filtCoef'));
      |   lowerLimit=Simulink.data.evalinGlobal(bdroot,get_param(gcb,'lowerLimit'));
      |   upperLimit=Simulink.data.evalinGlobal(bdroot,get_param(gcb,'upperLimit'));
      |   inscale=Simulink.data.evalinGlobal(bdroot,get_param(gcb,'inscale'));
      |   outscale=Simulink.data.evalinGlobal(bdroot,get_param(gcb,'outscale'));
      |   if (upperLimit<=lowerLimit)
      |     warning('UpperLimit should be greater than LowerLimit.');
      |   end
      |   if (inscale<=0)
      |     warning('E_max must be positive.');
      |   end
      |   if (outscale<=0)
      |     warning('U_max must be positive.');
      |   end
      |   kpf=pgain*inscale/outscale;
      |   s16PropGainShift=ceil(log2(abs(kpf)));
      |   if s16PropGainShift<-15
      |     s16PropGainShift=-15;
      |   end
      |   if s16PropGainShift>15
      |     s16PropGainShift=15;
      |     warning(['Parameter s16PropGainShift of ' gcb ' exceeds the fixed-point range.']);
      |   end
      |   f16PropGain=round(kpf*2^(-s16PropGainShift)*2^15);
      |   if f16PropGain>2^15-1
      |     f16PropGain=2^15-1;
      |     warning(['Parameter f16PropGain of ' gcb ' exceeds the fixed-point range.']);
      |   end
      |   if f16PropGain<-2^15
      |     f16PropGain=-2^15;
      |     warning(['Parameter f16PropGain of ' gcb ' exceeds the fixed-point range.']);
      |   end
      |   kif=igain*SampleTime*0.5*inscale/outscale;
      |   s16IntegGainShift=ceil(log2(abs(kif)));
      |   if s16IntegGainShift<-15
      |     s16IntegGainShift=-15;
      |   end
      |   if s16IntegGainShift>15
      |     s16IntegGainShift=15;
      |     warning(['Parameter s16IntegGainShift of ' gcb ' exceeds the fixed-point range.']);
      |   end
      |   f16IntegGain=round(kif*2^(-s16IntegGainShift)*2^15);
      |   if f16IntegGain>2^15-1
      |     f16IntegGain=2^15-1;
      |     warning(['Parameter f16IntegGain of ' gcb ' exceeds the fixed-point range.']);
      |   end
      |   if f16IntegGain<-2^15
      |     f16IntegGain=-2^15;
      |     warning(['Parameter f16IntegGain of ' gcb ' exceeds the fixed-point range.']);
      |   end
      |   upperLimitf=upperLimit/outscale;
      |   lowerLimitf=lowerLimit/outscale;
      |   f16UpperLimit=round(upperLimitf*2^15);
      |   if f16UpperLimit>2^15-1
      |     f16UpperLimit=2^15-1;
      |     warning(['Parameter f16UpperLimit of ' gcb ' exceeds the fixed-point range.']);
      |   end
      |   if f16UpperLimit<-2^15
      |     f16UpperLimit=-2^15;
      |     warning(['Parameter f16UpperLimit of ' gcb ' exceeds the fixed-point range.']);
      |   end
      |   f16LowerLimit=round(lowerLimitf*2^15);
      |   if f16LowerLimit>2^15-1
      |     f16LowerLimit=2^15-1;
      |     warning(['Parameter f16LowerLimit of ' gcb ' exceeds the fixed-point range.']);
      |   end
      |   if f16LowerLimit<-2^15
      |     f16LowerLimit=-2^15;
      |     warning(['Parameter f16LowerLimit of ' gcb ' exceeds the fixed-point range.']);
      |   end
      |   exparg=-SampleTime*filtCoef;
      |   expconst=exp(exparg);
      |   f16FiltCoef=round(expconst*2^15);
      |   if f16FiltCoef>2^15-1
      |     f16FiltCoef=2^15-1;
      |     warning(['Parameter f16FiltCoef of ' gcb ' exceeds the fixed-point range.']);
      |   end
      |   if f16FiltCoef<-2^15
      |     f16FiltCoef=-2^15;
      |     warning(['Parameter f16FiltCoef of ' gcb ' exceeds the fixed-point range.']);
      |   end
      |   kdf=dgain/SampleTime*(1 - expconst)*inscale/outscale;
      |   s16DerivGainShift=ceil(log2(abs(kpf)));
      |   if s16DerivGainShift<-15
      |     s16DerivGainShift=-15;
      |   end
      |   if s16DerivGainShift>15
      |     s16DerivGainShift=15;
      |     warning(['Parameter s16DerivGainShift of ' gcb ' exceeds the fixed-point range.']);
      |   end
      |   f16DerivGain=round(kpf*2^(-s16DerivGainShift)*2^15);
      |   if f16DerivGain>2^15-1
      |     f16DerivGain=2^15-1;
      |     warning(['Parameter f16DerivGain of ' gcb ' exceeds the fixed-point range.']);
      |   end
      |   if f16DerivGain<-2^15
      |     f16DerivGain=-2^15;
      |     warning(['Parameter f16DerivGain of ' gcb ' exceeds the fixed-point range.']);
      |   end
      |   if isnan(f16PropGain)
      |     if ~strcmp(f16PropGain_bkup,'0')
      |       set_param(gcb,'f16PropGain','0');
      |     end
      |   else
      |     tmps=num2str(f16PropGain);
      |     if ~strcmp(f16PropGain_bkup,tmps)
      |       set_param(gcb,'f16PropGain',tmps);
      |     end
      |   end
      |   if isnan(f16IntegGain)
      |     if ~strcmp(f16IntegGain_bkup,'0')
      |       set_param(gcb,'f16IntegGain','0');
      |     end
      |   else
      |     tmps=num2str(f16IntegGain);
      |     if ~strcmp(f16IntegGain_bkup,tmps)
      |       set_param(gcb,'f16IntegGain',tmps);
      |     end
      |   end
      |   if isnan(f16DerivGain)
      |     if ~strcmp(f16DerivGain_bkup,'0')
      |       set_param(gcb,'f16DerivGain','0');
      |     end
      |   else
      |     tmps=num2str(f16DerivGain);
      |     if ~strcmp(f16DerivGain_bkup,tmps)
      |       set_param(gcb,'f16DerivGain',tmps);
      |     end
      |   end
      |   if isnan(f16FiltCoef)
      |     if ~strcmp(f16FiltCoef_bkup,'0')
      |       set_param(gcb,'f16FiltCoef','0');
      |     end
      |   else
      |     tmps=num2str(f16FiltCoef);
      |     if ~strcmp(f16FiltCoef_bkup,tmps)
      |       set_param(gcb,'f16FiltCoef',tmps);
      |     end
      |   end
      |   if isnan(s16PropGainShift)
      |     if ~strcmp(s16PropGainShift_bkup,'0')
      |       set_param(gcb,'s16PropGainShift','0');
      |     end
      |   else
      |     tmps=num2str(s16PropGainShift);
      |     if ~strcmp(s16PropGainShift_bkup,tmps)
      |       set_param(gcb,'s16PropGainShift',tmps);
      |     end
      |   end
      |   if isnan(s16IntegGainShift)
      |     if ~strcmp(s16IntegGainShift_bkup,'0')
      |       set_param(gcb,'s16IntegGainShift','0');
      |     end
      |   else
      |     tmps=num2str(s16IntegGainShift);
      |     if ~strcmp(s16IntegGainShift_bkup,tmps)
      |       set_param(gcb,'s16IntegGainShift',tmps);
      |     end
      |   end
      |   if isnan(s16DerivGainShift)
      |     if ~strcmp(s16DerivGainShift_bkup,'0')
      |       set_param(gcb,'s16DerivGainShift','0');
      |     end
      |   else
      |     tmps=num2str(s16DerivGainShift);
      |     if ~strcmp(s16DerivGainShift_bkup,tmps)
      |       set_param(gcb,'s16DerivGainShift',tmps);
      |     end
      |   end
      |   if isnan(f16LowerLimit)
      |     if ~strcmp(f16LowerLimit_bkup,'0')
      |       set_param(gcb,'f16LowerLimit','0');
      |     end
      |   else
      |     tmps=num2str(f16LowerLimit);
      |     if ~strcmp(f16LowerLimit_bkup,tmps)
      |       set_param(gcb,'f16LowerLimit',tmps);
      |     end
      |   end
      |   if isnan(f16UpperLimit)
      |     if ~strcmp(f16UpperLimit_bkup,'0')
      |       set_param(gcb,'f16UpperLimit','0');
      |     end
      |   else
      |     tmps=num2str(f16UpperLimit);
      |     if ~strcmp(f16UpperLimit_bkup,tmps)
      |       set_param(gcb,'f16UpperLimit',tmps);
      |     end
      |   end
      | end
      mask Callback inscale:
      | autoCalcEn=get_param(gcb,'autoCalcEn');
      | if strcmp(autoCalcEn,'on')
      |   SampleTime=Simulink.data.evalinGlobal(bdroot,get_param(gcb,'SampleTime'));
      |   if (SampleTime==-1)
      |     SampleTime=str2double(get_param(gcb,'SampleTime_1'));
      |   end
      |   f16PropGain_bkup=get_param(gcb,'f16PropGain');
      |   f16IntegGain_bkup=get_param(gcb,'f16IntegGain');
      |   f16DerivGain_bkup=get_param(gcb,'f16DerivGain');
      |   f16FiltCoef_bkup=get_param(gcb,'f16FiltCoef');
      |   s16PropGainShift_bkup=get_param(gcb,'s16PropGainShift');
      |   s16IntegGainShift_bkup=get_param(gcb,'s16IntegGainShift');
      |   s16DerivGainShift_bkup=get_param(gcb,'s16DerivGainShift');
      |   f16LowerLimit_bkup=get_param(gcb,'f16LowerLimit');
      |   f16UpperLimit_bkup=get_param(gcb,'f16UpperLimit');
      |   pgain=Simulink.data.evalinGlobal(bdroot,get_param(gcb,'pgain'));
      |   igain=Simulink.data.evalinGlobal(bdroot,get_param(gcb,'igain'));
      |   dgain=Simulink.data.evalinGlobal(bdroot,get_param(gcb,'dgain'));
      |   filtCoef=Simulink.data.evalinGlobal(bdroot,get_param(gcb,'filtCoef'));
      |   lowerLimit=Simulink.data.evalinGlobal(bdroot,get_param(gcb,'lowerLimit'));
      |   upperLimit=Simulink.data.evalinGlobal(bdroot,get_param(gcb,'upperLimit'));
      |   inscale=Simulink.data.evalinGlobal(bdroot,get_param(gcb,'inscale'));
      |   outscale=Simulink.data.evalinGlobal(bdroot,get_param(gcb,'outscale'));
      |   if (upperLimit<=lowerLimit)
      |     warning('UpperLimit should be greater than LowerLimit.');
      |   end
      |   if (inscale<=0)
      |     warning('E_max must be positive.');
      |   end
      |   if (outscale<=0)
      |     warning('U_max must be positive.');
      |   end
      |   kpf=pgain*inscale/outscale;
      |   s16PropGainShift=ceil(log2(abs(kpf)));
      |   if s16PropGainShift<-15
      |     s16PropGainShift=-15;
      |   end
      |   if s16PropGainShift>15
      |     s16PropGainShift=15;
      |     warning(['Parameter s16PropGainShift of ' gcb ' exceeds the fixed-point range.']);
      |   end
      |   f16PropGain=round(kpf*2^(-s16PropGainShift)*2^15);
      |   if f16PropGain>2^15-1
      |     f16PropGain=2^15-1;
      |     warning(['Parameter f16PropGain of ' gcb ' exceeds the fixed-point range.']);
      |   end
      |   if f16PropGain<-2^15
      |     f16PropGain=-2^15;
      |     warning(['Parameter f16PropGain of ' gcb ' exceeds the fixed-point range.']);
      |   end
      |   kif=igain*SampleTime*0.5*inscale/outscale;
      |   s16IntegGainShift=ceil(log2(abs(kif)));
      |   if s16IntegGainShift<-15
      |     s16IntegGainShift=-15;
      |   end
      |   if s16IntegGainShift>15
      |     s16IntegGainShift=15;
      |     warning(['Parameter s16IntegGainShift of ' gcb ' exceeds the fixed-point range.']);
      |   end
      |   f16IntegGain=round(kif*2^(-s16IntegGainShift)*2^15);
      |   if f16IntegGain>2^15-1
      |     f16IntegGain=2^15-1;
      |     warning(['Parameter f16IntegGain of ' gcb ' exceeds the fixed-point range.']);
      |   end
      |   if f16IntegGain<-2^15
      |     f16IntegGain=-2^15;
      |     warning(['Parameter f16IntegGain of ' gcb ' exceeds the fixed-point range.']);
      |   end
      |   upperLimitf=upperLimit/outscale;
      |   lowerLimitf=lowerLimit/outscale;
      |   f16UpperLimit=round(upperLimitf*2^15);
      |   if f16UpperLimit>2^15-1
      |     f16UpperLimit=2^15-1;
      |     warning(['Parameter f16UpperLimit of ' gcb ' exceeds the fixed-point range.']);
      |   end
      |   if f16UpperLimit<-2^15
      |     f16UpperLimit=-2^15;
      |     warning(['Parameter f16UpperLimit of ' gcb ' exceeds the fixed-point range.']);
      |   end
      |   f16LowerLimit=round(lowerLimitf*2^15);
      |   if f16LowerLimit>2^15-1
      |     f16LowerLimit=2^15-1;
      |     warning(['Parameter f16LowerLimit of ' gcb ' exceeds the fixed-point range.']);
      |   end
      |   if f16LowerLimit<-2^15
      |     f16LowerLimit=-2^15;
      |     warning(['Parameter f16LowerLimit of ' gcb ' exceeds the fixed-point range.']);
      |   end
      |   exparg=-SampleTime*filtCoef;
      |   expconst=exp(exparg);
      |   f16FiltCoef=round(expconst*2^15);
      |   if f16FiltCoef>2^15-1
      |     f16FiltCoef=2^15-1;
      |     warning(['Parameter f16FiltCoef of ' gcb ' exceeds the fixed-point range.']);
      |   end
      |   if f16FiltCoef<-2^15
      |     f16FiltCoef=-2^15;
      |     warning(['Parameter f16FiltCoef of ' gcb ' exceeds the fixed-point range.']);
      |   end
      |   kdf=dgain/SampleTime*(1 - expconst)*inscale/outscale;
      |   s16DerivGainShift=ceil(log2(abs(kpf)));
      |   if s16DerivGainShift<-15
      |     s16DerivGainShift=-15;
      |   end
      |   if s16DerivGainShift>15
      |     s16DerivGainShift=15;
      |     warning(['Parameter s16DerivGainShift of ' gcb ' exceeds the fixed-point range.']);
      |   end
      |   f16DerivGain=round(kpf*2^(-s16DerivGainShift)*2^15);
      |   if f16DerivGain>2^15-1
      |     f16DerivGain=2^15-1;
      |     warning(['Parameter f16DerivGain of ' gcb ' exceeds the fixed-point range.']);
      |   end
      |   if f16DerivGain<-2^15
      |     f16DerivGain=-2^15;
      |     warning(['Parameter f16DerivGain of ' gcb ' exceeds the fixed-point range.']);
      |   end
      |   if isnan(f16PropGain)
      |     if ~strcmp(f16PropGain_bkup,'0')
      |       set_param(gcb,'f16PropGain','0');
      |     end
      |   else
      |     tmps=num2str(f16PropGain);
      |     if ~strcmp(f16PropGain_bkup,tmps)
      |       set_param(gcb,'f16PropGain',tmps);
      |     end
      |   end
      |   if isnan(f16IntegGain)
      |     if ~strcmp(f16IntegGain_bkup,'0')
      |       set_param(gcb,'f16IntegGain','0');
      |     end
      |   else
      |     tmps=num2str(f16IntegGain);
      |     if ~strcmp(f16IntegGain_bkup,tmps)
      |       set_param(gcb,'f16IntegGain',tmps);
      |     end
      |   end
      |   if isnan(f16DerivGain)
      |     if ~strcmp(f16DerivGain_bkup,'0')
      |       set_param(gcb,'f16DerivGain','0');
      |     end
      |   else
      |     tmps=num2str(f16DerivGain);
      |     if ~strcmp(f16DerivGain_bkup,tmps)
      |       set_param(gcb,'f16DerivGain',tmps);
      |     end
      |   end
      |   if isnan(f16FiltCoef)
      |     if ~strcmp(f16FiltCoef_bkup,'0')
      |       set_param(gcb,'f16FiltCoef','0');
      |     end
      |   else
      |     tmps=num2str(f16FiltCoef);
      |     if ~strcmp(f16FiltCoef_bkup,tmps)
      |       set_param(gcb,'f16FiltCoef',tmps);
      |     end
      |   end
      |   if isnan(s16PropGainShift)
      |     if ~strcmp(s16PropGainShift_bkup,'0')
      |       set_param(gcb,'s16PropGainShift','0');
      |     end
      |   else
      |     tmps=num2str(s16PropGainShift);
      |     if ~strcmp(s16PropGainShift_bkup,tmps)
      |       set_param(gcb,'s16PropGainShift',tmps);
      |     end
      |   end
      |   if isnan(s16IntegGainShift)
      |     if ~strcmp(s16IntegGainShift_bkup,'0')
      |       set_param(gcb,'s16IntegGainShift','0');
      |     end
      |   else
      |     tmps=num2str(s16IntegGainShift);
      |     if ~strcmp(s16IntegGainShift_bkup,tmps)
      |       set_param(gcb,'s16IntegGainShift',tmps);
      |     end
      |   end
      |   if isnan(s16DerivGainShift)
      |     if ~strcmp(s16DerivGainShift_bkup,'0')
      |       set_param(gcb,'s16DerivGainShift','0');
      |     end
      |   else
      |     tmps=num2str(s16DerivGainShift);
      |     if ~strcmp(s16DerivGainShift_bkup,tmps)
      |       set_param(gcb,'s16DerivGainShift',tmps);
      |     end
      |   end
      |   if isnan(f16LowerLimit)
      |     if ~strcmp(f16LowerLimit_bkup,'0')
      |       set_param(gcb,'f16LowerLimit','0');
      |     end
      |   else
      |     tmps=num2str(f16LowerLimit);
      |     if ~strcmp(f16LowerLimit_bkup,tmps)
      |       set_param(gcb,'f16LowerLimit',tmps);
      |     end
      |   end
      |   if isnan(f16UpperLimit)
      |     if ~strcmp(f16UpperLimit_bkup,'0')
      |       set_param(gcb,'f16UpperLimit','0');
      |     end
      |   else
      |     tmps=num2str(f16UpperLimit);
      |     if ~strcmp(f16UpperLimit_bkup,tmps)
      |       set_param(gcb,'f16UpperLimit',tmps);
      |     end
      |   end
      | end
      mask Callback outscale:
      | autoCalcEn=get_param(gcb,'autoCalcEn');
      | if strcmp(autoCalcEn,'on')
      |   SampleTime=Simulink.data.evalinGlobal(bdroot,get_param(gcb,'SampleTime'));
      |   if (SampleTime==-1)
      |     SampleTime=str2double(get_param(gcb,'SampleTime_1'));
      |   end
      |   f16PropGain_bkup=get_param(gcb,'f16PropGain');
      |   f16IntegGain_bkup=get_param(gcb,'f16IntegGain');
      |   f16DerivGain_bkup=get_param(gcb,'f16DerivGain');
      |   f16FiltCoef_bkup=get_param(gcb,'f16FiltCoef');
      |   s16PropGainShift_bkup=get_param(gcb,'s16PropGainShift');
      |   s16IntegGainShift_bkup=get_param(gcb,'s16IntegGainShift');
      |   s16DerivGainShift_bkup=get_param(gcb,'s16DerivGainShift');
      |   f16LowerLimit_bkup=get_param(gcb,'f16LowerLimit');
      |   f16UpperLimit_bkup=get_param(gcb,'f16UpperLimit');
      |   pgain=Simulink.data.evalinGlobal(bdroot,get_param(gcb,'pgain'));
      |   igain=Simulink.data.evalinGlobal(bdroot,get_param(gcb,'igain'));
      |   dgain=Simulink.data.evalinGlobal(bdroot,get_param(gcb,'dgain'));
      |   filtCoef=Simulink.data.evalinGlobal(bdroot,get_param(gcb,'filtCoef'));
      |   lowerLimit=Simulink.data.evalinGlobal(bdroot,get_param(gcb,'lowerLimit'));
      |   upperLimit=Simulink.data.evalinGlobal(bdroot,get_param(gcb,'upperLimit'));
      |   inscale=Simulink.data.evalinGlobal(bdroot,get_param(gcb,'inscale'));
      |   outscale=Simulink.data.evalinGlobal(bdroot,get_param(gcb,'outscale'));
      |   if (upperLimit<=lowerLimit)
      |     warning('UpperLimit should be greater than LowerLimit.');
      |   end
      |   if (inscale<=0)
      |     warning('E_max must be positive.');
      |   end
      |   if (outscale<=0)
      |     warning('U_max must be positive.');
      |   end
      |   kpf=pgain*inscale/outscale;
      |   s16PropGainShift=ceil(log2(abs(kpf)));
      |   if s16PropGainShift<-15
      |     s16PropGainShift=-15;
      |   end
      |   if s16PropGainShift>15
      |     s16PropGainShift=15;
      |     warning(['Parameter s16PropGainShift of ' gcb ' exceeds the fixed-point range.']);
      |   end
      |   f16PropGain=round(kpf*2^(-s16PropGainShift)*2^15);
      |   if f16PropGain>2^15-1
      |     f16PropGain=2^15-1;
      |     warning(['Parameter f16PropGain of ' gcb ' exceeds the fixed-point range.']);
      |   end
      |   if f16PropGain<-2^15
      |     f16PropGain=-2^15;
      |     warning(['Parameter f16PropGain of ' gcb ' exceeds the fixed-point range.']);
      |   end
      |   kif=igain*SampleTime*0.5*inscale/outscale;
      |   s16IntegGainShift=ceil(log2(abs(kif)));
      |   if s16IntegGainShift<-15
      |     s16IntegGainShift=-15;
      |   end
      |   if s16IntegGainShift>15
      |     s16IntegGainShift=15;
      |     warning(['Parameter s16IntegGainShift of ' gcb ' exceeds the fixed-point range.']);
      |   end
      |   f16IntegGain=round(kif*2^(-s16IntegGainShift)*2^15);
      |   if f16IntegGain>2^15-1
      |     f16IntegGain=2^15-1;
      |     warning(['Parameter f16IntegGain of ' gcb ' exceeds the fixed-point range.']);
      |   end
      |   if f16IntegGain<-2^15
      |     f16IntegGain=-2^15;
      |     warning(['Parameter f16IntegGain of ' gcb ' exceeds the fixed-point range.']);
      |   end
      |   upperLimitf=upperLimit/outscale;
      |   lowerLimitf=lowerLimit/outscale;
      |   f16UpperLimit=round(upperLimitf*2^15);
      |   if f16UpperLimit>2^15-1
      |     f16UpperLimit=2^15-1;
      |     warning(['Parameter f16UpperLimit of ' gcb ' exceeds the fixed-point range.']);
      |   end
      |   if f16UpperLimit<-2^15
      |     f16UpperLimit=-2^15;
      |     warning(['Parameter f16UpperLimit of ' gcb ' exceeds the fixed-point range.']);
      |   end
      |   f16LowerLimit=round(lowerLimitf*2^15);
      |   if f16LowerLimit>2^15-1
      |     f16LowerLimit=2^15-1;
      |     warning(['Parameter f16LowerLimit of ' gcb ' exceeds the fixed-point range.']);
      |   end
      |   if f16LowerLimit<-2^15
      |     f16LowerLimit=-2^15;
      |     warning(['Parameter f16LowerLimit of ' gcb ' exceeds the fixed-point range.']);
      |   end
      |   exparg=-SampleTime*filtCoef;
      |   expconst=exp(exparg);
      |   f16FiltCoef=round(expconst*2^15);
      |   if f16FiltCoef>2^15-1
      |     f16FiltCoef=2^15-1;
      |     warning(['Parameter f16FiltCoef of ' gcb ' exceeds the fixed-point range.']);
      |   end
      |   if f16FiltCoef<-2^15
      |     f16FiltCoef=-2^15;
      |     warning(['Parameter f16FiltCoef of ' gcb ' exceeds the fixed-point range.']);
      |   end
      |   kdf=dgain/SampleTime*(1 - expconst)*inscale/outscale;
      |   s16DerivGainShift=ceil(log2(abs(kpf)));
      |   if s16DerivGainShift<-15
      |     s16DerivGainShift=-15;
      |   end
      |   if s16DerivGainShift>15
      |     s16DerivGainShift=15;
      |     warning(['Parameter s16DerivGainShift of ' gcb ' exceeds the fixed-point range.']);
      |   end
      |   f16DerivGain=round(kpf*2^(-s16DerivGainShift)*2^15);
      |   if f16DerivGain>2^15-1
      |     f16DerivGain=2^15-1;
      |     warning(['Parameter f16DerivGain of ' gcb ' exceeds the fixed-point range.']);
      |   end
      |   if f16DerivGain<-2^15
      |     f16DerivGain=-2^15;
      |     warning(['Parameter f16DerivGain of ' gcb ' exceeds the fixed-point range.']);
      |   end
      |   if isnan(f16PropGain)
      |     if ~strcmp(f16PropGain_bkup,'0')
      |       set_param(gcb,'f16PropGain','0');
      |     end
      |   else
      |     tmps=num2str(f16PropGain);
      |     if ~strcmp(f16PropGain_bkup,tmps)
      |       set_param(gcb,'f16PropGain',tmps);
      |     end
      |   end
      |   if isnan(f16IntegGain)
      |     if ~strcmp(f16IntegGain_bkup,'0')
      |       set_param(gcb,'f16IntegGain','0');
      |     end
      |   else
      |     tmps=num2str(f16IntegGain);
      |     if ~strcmp(f16IntegGain_bkup,tmps)
      |       set_param(gcb,'f16IntegGain',tmps);
      |     end
      |   end
      |   if isnan(f16DerivGain)
      |     if ~strcmp(f16DerivGain_bkup,'0')
      |       set_param(gcb,'f16DerivGain','0');
      |     end
      |   else
      |     tmps=num2str(f16DerivGain);
      |     if ~strcmp(f16DerivGain_bkup,tmps)
      |       set_param(gcb,'f16DerivGain',tmps);
      |     end
      |   end
      |   if isnan(f16FiltCoef)
      |     if ~strcmp(f16FiltCoef_bkup,'0')
      |       set_param(gcb,'f16FiltCoef','0');
      |     end
      |   else
      |     tmps=num2str(f16FiltCoef);
      |     if ~strcmp(f16FiltCoef_bkup,tmps)
      |       set_param(gcb,'f16FiltCoef',tmps);
      |     end
      |   end
      |   if isnan(s16PropGainShift)
      |     if ~strcmp(s16PropGainShift_bkup,'0')
      |       set_param(gcb,'s16PropGainShift','0');
      |     end
      |   else
      |     tmps=num2str(s16PropGainShift);
      |     if ~strcmp(s16PropGainShift_bkup,tmps)
      |       set_param(gcb,'s16PropGainShift',tmps);
      |     end
      |   end
      |   if isnan(s16IntegGainShift)
      |     if ~strcmp(s16IntegGainShift_bkup,'0')
      |       set_param(gcb,'s16IntegGainShift','0');
      |     end
      |   else
      |     tmps=num2str(s16IntegGainShift);
      |     if ~strcmp(s16IntegGainShift_bkup,tmps)
      |       set_param(gcb,'s16IntegGainShift',tmps);
      |     end
      |   end
      |   if isnan(s16DerivGainShift)
      |     if ~strcmp(s16DerivGainShift_bkup,'0')
      |       set_param(gcb,'s16DerivGainShift','0');
      |     end
      |   else
      |     tmps=num2str(s16DerivGainShift);
      |     if ~strcmp(s16DerivGainShift_bkup,tmps)
      |       set_param(gcb,'s16DerivGainShift',tmps);
      |     end
      |   end
      |   if isnan(f16LowerLimit)
      |     if ~strcmp(f16LowerLimit_bkup,'0')
      |       set_param(gcb,'f16LowerLimit','0');
      |     end
      |   else
      |     tmps=num2str(f16LowerLimit);
      |     if ~strcmp(f16LowerLimit_bkup,tmps)
      |       set_param(gcb,'f16LowerLimit',tmps);
      |     end
      |   end
      |   if isnan(f16UpperLimit)
      |     if ~strcmp(f16UpperLimit_bkup,'0')
      |       set_param(gcb,'f16UpperLimit','0');
      |     end
      |   else
      |     tmps=num2str(f16UpperLimit);
      |     if ~strcmp(f16UpperLimit_bkup,tmps)
      |       set_param(gcb,'f16UpperLimit',tmps);
      |     end
      |   end
      | end
      mask Callback autoCalcEn:
      | maskStr=get_param(gcb,'showStates');
      | if strcmp(maskStr,'Hide (faster execution)')
      |   p=Simulink.Mask.get(gcb);
      |   autoCalcEn=get_param(gcb,'autoCalcEn');
      |   hintText=p.getDialogControl('timeHint');
      |   if strcmp(autoCalcEn,'on')
      |     param=p.getParameter('outscale');
      |     if strcmp(param.Enabled,'off')
      |       SampleTime=Simulink.data.evalinGlobal(bdroot,get_param(gcb,'SampleTime'));
      |       if SampleTime==-1
      |         SampleTime=str2double(get_param(gcb,'SampleTime_1'));
      |         if isnan(SampleTime)
      |           hintText.Prompt=['Note: Implementation parameters cannot be calculated yet because the block''s inherited sample time is unknown. Simulink will update the sample time when you run the simulation.'];
      |         else
      |           hintText.Prompt=['Caution: Implementation parameters depend on inherited sample time. Make sure that the sample time of the block''s inputs corresponds to the sampling period in the target application.'];
      |         end
      |       else
      |         hintText.Prompt='Caution: Implementation parameters depend on the sample time. Make sure that the simulation time step corresponds to the sampling period in the target application.';
      |       end
      |       p=Simulink.Mask.get(gcb);
      |       param=p.getParameter('pgain');
      |       param.set('Enabled','on');
      |       param=p.getParameter('igain');
      |       param.set('Enabled','on');
      |       param=p.getParameter('dgain');
      |       param.set('Enabled','on');
      |       param=p.getParameter('filtCoef');
      |       param.set('Enabled','on');
      |       param=p.getParameter('lowerLimit');
      |       param.set('Enabled','on');
      |       param=p.getParameter('upperLimit');
      |       param.set('Enabled','on');
      |       param=p.getParameter('inscale');
      |       param.set('Enabled','on');
      |       param=p.getParameter('outscale');
      |       param.set('Enabled','on');
      |     else
      |       SampleTime=Simulink.data.evalinGlobal(bdroot,get_param(gcb,'SampleTime'));
      |       if SampleTime==-1
      |         SampleTime=str2double(get_param(gcb,'SampleTime_1'));
      |       end
      |     end
      |     f16PropGain_bkup=get_param(gcb,'f16PropGain');
      |     f16IntegGain_bkup=get_param(gcb,'f16IntegGain');
      |     f16DerivGain_bkup=get_param(gcb,'f16DerivGain');
      |     f16FiltCoef_bkup=get_param(gcb,'f16FiltCoef');
      |     s16PropGainShift_bkup=get_param(gcb,'s16PropGainShift');
      |     s16IntegGainShift_bkup=get_param(gcb,'s16IntegGainShift');
      |     s16DerivGainShift_bkup=get_param(gcb,'s16DerivGainShift');
      |     f16LowerLimit_bkup=get_param(gcb,'f16LowerLimit');
      |     f16UpperLimit_bkup=get_param(gcb,'f16UpperLimit');
      |     pgain=Simulink.data.evalinGlobal(bdroot,get_param(gcb,'pgain'));
      |     igain=Simulink.data.evalinGlobal(bdroot,get_param(gcb,'igain'));
      |     dgain=Simulink.data.evalinGlobal(bdroot,get_param(gcb,'dgain'));
      |     filtCoef=Simulink.data.evalinGlobal(bdroot,get_param(gcb,'filtCoef'));
      |     lowerLimit=Simulink.data.evalinGlobal(bdroot,get_param(gcb,'lowerLimit'));
      |     upperLimit=Simulink.data.evalinGlobal(bdroot,get_param(gcb,'upperLimit'));
      |     inscale=Simulink.data.evalinGlobal(bdroot,get_param(gcb,'inscale'));
      |     outscale=Simulink.data.evalinGlobal(bdroot,get_param(gcb,'outscale'));
      |     if (upperLimit<=lowerLimit)
      |       warning('UpperLimit should be greater than LowerLimit.');
      |     end
      |     if (inscale<=0)
      |       warning('E_max must be positive.');
      |     end
      |     if (outscale<=0)
      |       warning('U_max must be positive.');
      |     end
      |     kpf=pgain*inscale/outscale;
      |     s16PropGainShift=ceil(log2(abs(kpf)));
      |     if s16PropGainShift<-15
      |       s16PropGainShift=-15;
      |     end
      |     if s16PropGainShift>15
      |       s16PropGainShift=15;
      |       warning(['Parameter s16PropGainShift of ' gcb ' exceeds the fixed-point range.']);
      |     end
      |     f16PropGain=round(kpf*2^(-s16PropGainShift)*2^15);
      |     if f16PropGain>2^15-1
      |       f16PropGain=2^15-1;
      |       warning(['Parameter f16PropGain of ' gcb ' exceeds the fixed-point range.']);
      |     end
      |     if f16PropGain<-2^15
      |       f16PropGain=-2^15;
      |       warning(['Parameter f16PropGain of ' gcb ' exceeds the fixed-point range.']);
      |     end
      |     kif=igain*SampleTime*0.5*inscale/outscale;
      |     s16IntegGainShift=ceil(log2(abs(kif)));
      |     if s16IntegGainShift<-15
      |       s16IntegGainShift=-15;
      |     end
      |     if s16IntegGainShift>15
      |       s16IntegGainShift=15;
      |       warning(['Parameter s16IntegGainShift of ' gcb ' exceeds the fixed-point range.']);
      |     end
      |     f16IntegGain=round(kif*2^(-s16IntegGainShift)*2^15);
      |     if f16IntegGain>2^15-1
      |       f16IntegGain=2^15-1;
      |       warning(['Parameter f16IntegGain of ' gcb ' exceeds the fixed-point range.']);
      |     end
      |     if f16IntegGain<-2^15
      |       f16IntegGain=-2^15;
      |       warning(['Parameter f16IntegGain of ' gcb ' exceeds the fixed-point range.']);
      |     end
      |     upperLimitf=upperLimit/outscale;
      |     lowerLimitf=lowerLimit/outscale;
      |     f16UpperLimit=round(upperLimitf*2^15);
      |     if f16UpperLimit>2^15-1
      |       f16UpperLimit=2^15-1;
      |       warning(['Parameter f16UpperLimit of ' gcb ' exceeds the fixed-point range.']);
      |     end
      |     if f16UpperLimit<-2^15
      |       f16UpperLimit=-2^15;
      |       warning(['Parameter f16UpperLimit of ' gcb ' exceeds the fixed-point range.']);
      |     end
      |     f16LowerLimit=round(lowerLimitf*2^15);
      |     if f16LowerLimit>2^15-1
      |       f16LowerLimit=2^15-1;
      |       warning(['Parameter f16LowerLimit of ' gcb ' exceeds the fixed-point range.']);
      |     end
      |     if f16LowerLimit<-2^15
      |       f16LowerLimit=-2^15;
      |       warning(['Parameter f16LowerLimit of ' gcb ' exceeds the fixed-point range.']);
      |     end
      |     exparg=-SampleTime*filtCoef;
      |     expconst=exp(exparg);
      |     f16FiltCoef=round(expconst*2^15);
      |     if f16FiltCoef>2^15-1
      |       f16FiltCoef=2^15-1;
      |       warning(['Parameter f16FiltCoef of ' gcb ' exceeds the fixed-point range.']);
      |     end
      |     if f16FiltCoef<-2^15
      |       f16FiltCoef=-2^15;
      |       warning(['Parameter f16FiltCoef of ' gcb ' exceeds the fixed-point range.']);
      |     end
      |     kdf=dgain/SampleTime*(1 - expconst)*inscale/outscale;
      |     s16DerivGainShift=ceil(log2(abs(kpf)));
      |     if s16DerivGainShift<-15
      |       s16DerivGainShift=-15;
      |     end
      |     if s16DerivGainShift>15
      |       s16DerivGainShift=15;
      |       warning(['Parameter s16DerivGainShift of ' gcb ' exceeds the fixed-point range.']);
      |     end
      |     f16DerivGain=round(kpf*2^(-s16DerivGainShift)*2^15);
      |     if f16DerivGain>2^15-1
      |       f16DerivGain=2^15-1;
      |       warning(['Parameter f16DerivGain of ' gcb ' exceeds the fixed-point range.']);
      |     end
      |     if f16DerivGain<-2^15
      |       f16DerivGain=-2^15;
      |       warning(['Parameter f16DerivGain of ' gcb ' exceeds the fixed-point range.']);
      |     end
      |     if isnan(f16PropGain)
      |       if ~strcmp(f16PropGain_bkup,'0')
      |         set_param(gcb,'f16PropGain','0');
      |       end
      |     else
      |       tmps=num2str(f16PropGain);
      |       if ~strcmp(f16PropGain_bkup,tmps)
      |         set_param(gcb,'f16PropGain',tmps);
      |       end
      |     end
      |     if isnan(f16IntegGain)
      |       if ~strcmp(f16IntegGain_bkup,'0')
      |         set_param(gcb,'f16IntegGain','0');
      |       end
      |     else
      |       tmps=num2str(f16IntegGain);
      |       if ~strcmp(f16IntegGain_bkup,tmps)
      |         set_param(gcb,'f16IntegGain',tmps);
      |       end
      |     end
      |     if isnan(f16DerivGain)
      |       if ~strcmp(f16DerivGain_bkup,'0')
      |         set_param(gcb,'f16DerivGain','0');
      |       end
      |     else
      |       tmps=num2str(f16DerivGain);
      |       if ~strcmp(f16DerivGain_bkup,tmps)
      |         set_param(gcb,'f16DerivGain',tmps);
      |       end
      |     end
      |     if isnan(f16FiltCoef)
      |       if ~strcmp(f16FiltCoef_bkup,'0')
      |         set_param(gcb,'f16FiltCoef','0');
      |       end
      |     else
      |       tmps=num2str(f16FiltCoef);
      |       if ~strcmp(f16FiltCoef_bkup,tmps)
      |         set_param(gcb,'f16FiltCoef',tmps);
      |       end
      |     end
      |     if isnan(s16PropGainShift)
      |       if ~strcmp(s16PropGainShift_bkup,'0')
      |         set_param(gcb,'s16PropGainShift','0');
      |       end
      |     else
      |       tmps=num2str(s16PropGainShift);
      |       if ~strcmp(s16PropGainShift_bkup,tmps)
      |         set_param(gcb,'s16PropGainShift',tmps);
      |       end
      |     end
      |     if isnan(s16IntegGainShift)
      |       if ~strcmp(s16IntegGainShift_bkup,'0')
      |         set_param(gcb,'s16IntegGainShift','0');
      |       end
      |     else
      |       tmps=num2str(s16IntegGainShift);
      |       if ~strcmp(s16IntegGainShift_bkup,tmps)
      |         set_param(gcb,'s16IntegGainShift',tmps);
      |       end
      |     end
      |     if isnan(s16DerivGainShift)
      |       if ~strcmp(s16DerivGainShift_bkup,'0')
      |         set_param(gcb,'s16DerivGainShift','0');
      |       end
      |     else
      |       tmps=num2str(s16DerivGainShift);
      |       if ~strcmp(s16DerivGainShift_bkup,tmps)
      |         set_param(gcb,'s16DerivGainShift',tmps);
      |       end
      |     end
      |     if isnan(f16LowerLimit)
      |       if ~strcmp(f16LowerLimit_bkup,'0')
      |         set_param(gcb,'f16LowerLimit','0');
      |       end
      |     else
      |       tmps=num2str(f16LowerLimit);
      |       if ~strcmp(f16LowerLimit_bkup,tmps)
      |         set_param(gcb,'f16LowerLimit',tmps);
      |       end
      |     end
      |     if isnan(f16UpperLimit)
      |       if ~strcmp(f16UpperLimit_bkup,'0')
      |         set_param(gcb,'f16UpperLimit','0');
      |       end
      |     else
      |       tmps=num2str(f16UpperLimit);
      |       if ~strcmp(f16UpperLimit_bkup,tmps)
      |         set_param(gcb,'f16UpperLimit',tmps);
      |       end
      |     end
      |   else
      |     param=p.getParameter('outscale');
      |     if strcmp(param.Enabled,'on')
      |       hintText.Prompt='Caution: Implementation parameters are fixed.';
      |       p=Simulink.Mask.get(gcb);
      |       param=p.getParameter('pgain');
      |       param.set('Enabled','off');
      |       param=p.getParameter('igain');
      |       param.set('Enabled','off');
      |       param=p.getParameter('dgain');
      |       param.set('Enabled','off');
      |       param=p.getParameter('filtCoef');
      |       param.set('Enabled','off');
      |       param=p.getParameter('lowerLimit');
      |       param.set('Enabled','off');
      |       param=p.getParameter('upperLimit');
      |       param.set('Enabled','off');
      |       param=p.getParameter('inscale');
      |       param.set('Enabled','off');
      |       param=p.getParameter('outscale');
      |       param.set('Enabled','off');
      |     end
      |   end
      | end
      mask DialogControl CompBut Prompt: Recalculate sample times
      mask DialogControl CompBut Tooltip: Simulink updates the sample times of all blocks when the simulation is run. This button will update the sample times now.
      mask DialogControl CompBut Callback:
      | btn=questdlg('This will apply all changes in all open dialog boxes and update the schematic. Do you want to proceed?','Apply all changes','Continue','Cancel','Continue');
      | if strcmp(btn,'Continue')
      |   dlgs=DAStudio.ToolRoot.getOpenDialogs;
      |   for i=1:length(dlgs)
      |     dlgs(i).apply;
      |   end
      |   try
      |     SampleTime_1=str2double(get_param(gcb,'SampleTime_1'));
      |     ts=Simulink.Block.getSampleTimes(gcb);
      |     ts=ts(1).Value(1);
      |     if (SampleTime_1 ~= ts)
      |       SampleTime_1=ts;
      |       set_param(gcb,'SampleTime_1',num2str(ts));
      |       autoCalcEn=get_param(gcb,'autoCalcEn');
      |       if strcmp(autoCalcEn,'on')
      |         SampleTime=Simulink.data.evalinGlobal(bdroot,get_param(gcb,'SampleTime'));
      |         p=Simulink.Mask.get(gcb);
      |         hintText=p.getDialogControl('timeHint');
      |         if SampleTime==-1
      |           SampleTime=SampleTime_1;
      |           hintText.Prompt='Caution: Implementation parameters depend on inherited sample time. Make sure that the sample time of the block''s inputs corresponds to the sampling period in the target application.';
      |         else
      |           hintText.Prompt='Caution: Implementation parameters depend on the sample time. Make sure that the simulation time step corresponds to the sampling period in the target application.';
      |         end
      |         f16PropGain_bkup=get_param(gcb,'f16PropGain');
      |         f16IntegGain_bkup=get_param(gcb,'f16IntegGain');
      |         f16DerivGain_bkup=get_param(gcb,'f16DerivGain');
      |         f16FiltCoef_bkup=get_param(gcb,'f16FiltCoef');
      |         s16PropGainShift_bkup=get_param(gcb,'s16PropGainShift');
      |         s16IntegGainShift_bkup=get_param(gcb,'s16IntegGainShift');
      |         s16DerivGainShift_bkup=get_param(gcb,'s16DerivGainShift');
      |         f16LowerLimit_bkup=get_param(gcb,'f16LowerLimit');
      |         f16UpperLimit_bkup=get_param(gcb,'f16UpperLimit');
      |         pgain=Simulink.data.evalinGlobal(bdroot,get_param(gcb,'pgain'));
      |         igain=Simulink.data.evalinGlobal(bdroot,get_param(gcb,'igain'));
      |         dgain=Simulink.data.evalinGlobal(bdroot,get_param(gcb,'dgain'));
      |         filtCoef=Simulink.data.evalinGlobal(bdroot,get_param(gcb,'filtCoef'));
      |         lowerLimit=Simulink.data.evalinGlobal(bdroot,get_param(gcb,'lowerLimit'));
      |         upperLimit=Simulink.data.evalinGlobal(bdroot,get_param(gcb,'upperLimit'));
      |         inscale=Simulink.data.evalinGlobal(bdroot,get_param(gcb,'inscale'));
      |         outscale=Simulink.data.evalinGlobal(bdroot,get_param(gcb,'outscale'));
      |         if (upperLimit<=lowerLimit)
      |           warning('UpperLimit should be greater than LowerLimit.');
      |         end
      |         if (inscale<=0)
      |           warning('E_max must be positive.');
      |         end
      |         if (outscale<=0)
      |           warning('U_max must be positive.');
      |         end
      |         kpf=pgain*inscale/outscale;
      |         s16PropGainShift=ceil(log2(abs(kpf)));
      |         if s16PropGainShift<-15
      |           s16PropGainShift=-15;
      |         end
      |         if s16PropGainShift>15
      |           s16PropGainShift=15;
      |           warning(['Parameter s16PropGainShift of ' gcb ' exceeds the fixed-point range.']);
      |         end
      |         f16PropGain=round(kpf*2^(-s16PropGainShift)*2^15);
      |         if f16PropGain>2^15-1
      |           f16PropGain=2^15-1;
      |           warning(['Parameter f16PropGain of ' gcb ' exceeds the fixed-point range.']);
      |         end
      |         if f16PropGain<-2^15
      |           f16PropGain=-2^15;
      |           warning(['Parameter f16PropGain of ' gcb ' exceeds the fixed-point range.']);
      |         end
      |         kif=igain*SampleTime*0.5*inscale/outscale;
      |         s16IntegGainShift=ceil(log2(abs(kif)));
      |         if s16IntegGainShift<-15
      |           s16IntegGainShift=-15;
      |         end
      |         if s16IntegGainShift>15
      |           s16IntegGainShift=15;
      |           warning(['Parameter s16IntegGainShift of ' gcb ' exceeds the fixed-point range.']);
      |         end
      |         f16IntegGain=round(kif*2^(-s16IntegGainShift)*2^15);
      |         if f16IntegGain>2^15-1
      |           f16IntegGain=2^15-1;
      |           warning(['Parameter f16IntegGain of ' gcb ' exceeds the fixed-point range.']);
      |         end
      |         if f16IntegGain<-2^15
      |           f16IntegGain=-2^15;
      |           warning(['Parameter f16IntegGain of ' gcb ' exceeds the fixed-point range.']);
      |         end
      |         upperLimitf=upperLimit/outscale;
      |         lowerLimitf=lowerLimit/outscale;
      |         f16UpperLimit=round(upperLimitf*2^15);
      |         if f16UpperLimit>2^15-1
      |           f16UpperLimit=2^15-1;
      |           warning(['Parameter f16UpperLimit of ' gcb ' exceeds the fixed-point range.']);
      |         end
      |         if f16UpperLimit<-2^15
      |           f16UpperLimit=-2^15;
      |           warning(['Parameter f16UpperLimit of ' gcb ' exceeds the fixed-point range.']);
      |         end
      |         f16LowerLimit=round(lowerLimitf*2^15);
      |         if f16LowerLimit>2^15-1
      |           f16LowerLimit=2^15-1;
      |           warning(['Parameter f16LowerLimit of ' gcb ' exceeds the fixed-point range.']);
      |         end
      |         if f16LowerLimit<-2^15
      |           f16LowerLimit=-2^15;
      |           warning(['Parameter f16LowerLimit of ' gcb ' exceeds the fixed-point range.']);
      |         end
      |         exparg=-SampleTime*filtCoef;
      |         expconst=exp(exparg);
      |         f16FiltCoef=round(expconst*2^15);
      |         if f16FiltCoef>2^15-1
      |           f16FiltCoef=2^15-1;
      |           warning(['Parameter f16FiltCoef of ' gcb ' exceeds the fixed-point range.']);
      |         end
      |         if f16FiltCoef<-2^15
      |           f16FiltCoef=-2^15;
      |           warning(['Parameter f16FiltCoef of ' gcb ' exceeds the fixed-point range.']);
      |         end
      |         kdf=dgain/SampleTime*(1 - expconst)*inscale/outscale;
      |         s16DerivGainShift=ceil(log2(abs(kpf)));
      |         if s16DerivGainShift<-15
      |           s16DerivGainShift=-15;
      |         end
      |         if s16DerivGainShift>15
      |           s16DerivGainShift=15;
      |           warning(['Parameter s16DerivGainShift of ' gcb ' exceeds the fixed-point range.']);
      |         end
      |         f16DerivGain=round(kpf*2^(-s16DerivGainShift)*2^15);
      |         if f16DerivGain>2^15-1
      |           f16DerivGain=2^15-1;
      |           warning(['Parameter f16DerivGain of ' gcb ' exceeds the fixed-point range.']);
      |         end
      |         if f16DerivGain<-2^15
      |           f16DerivGain=-2^15;
      |           warning(['Parameter f16DerivGain of ' gcb ' exceeds the fixed-point range.']);
      |         end
      |         if isnan(f16PropGain)
      |           if ~strcmp(f16PropGain_bkup,'0')
      |             set_param(gcb,'f16PropGain','0');
      |           end
      |         else
      |           tmps=num2str(f16PropGain);
      |           if ~strcmp(f16PropGain_bkup,tmps)
      |             set_param(gcb,'f16PropGain',tmps);
      |           end
      |         end
      |         if isnan(f16IntegGain)
      |           if ~strcmp(f16IntegGain_bkup,'0')
      |             set_param(gcb,'f16IntegGain','0');
      |           end
      |         else
      |           tmps=num2str(f16IntegGain);
      |           if ~strcmp(f16IntegGain_bkup,tmps)
      |             set_param(gcb,'f16IntegGain',tmps);
      |           end
      |         end
      |         if isnan(f16DerivGain)
      |           if ~strcmp(f16DerivGain_bkup,'0')
      |             set_param(gcb,'f16DerivGain','0');
      |           end
      |         else
      |           tmps=num2str(f16DerivGain);
      |           if ~strcmp(f16DerivGain_bkup,tmps)
      |             set_param(gcb,'f16DerivGain',tmps);
      |           end
      |         end
      |         if isnan(f16FiltCoef)
      |           if ~strcmp(f16FiltCoef_bkup,'0')
      |             set_param(gcb,'f16FiltCoef','0');
      |           end
      |         else
      |           tmps=num2str(f16FiltCoef);
      |           if ~strcmp(f16FiltCoef_bkup,tmps)
      |             set_param(gcb,'f16FiltCoef',tmps);
      |           end
      |         end
      |         if isnan(s16PropGainShift)
      |           if ~strcmp(s16PropGainShift_bkup,'0')
      |             set_param(gcb,'s16PropGainShift','0');
      |           end
      |         else
      |           tmps=num2str(s16PropGainShift);
      |           if ~strcmp(s16PropGainShift_bkup,tmps)
      |             set_param(gcb,'s16PropGainShift',tmps);
      |           end
      |         end
      |         if isnan(s16IntegGainShift)
      |           if ~strcmp(s16IntegGainShift_bkup,'0')
      |             set_param(gcb,'s16IntegGainShift','0');
      |           end
      |         else
      |           tmps=num2str(s16IntegGainShift);
      |           if ~strcmp(s16IntegGainShift_bkup,tmps)
      |             set_param(gcb,'s16IntegGainShift',tmps);
      |           end
      |         end
      |         if isnan(s16DerivGainShift)
      |           if ~strcmp(s16DerivGainShift_bkup,'0')
      |             set_param(gcb,'s16DerivGainShift','0');
      |           end
      |         else
      |           tmps=num2str(s16DerivGainShift);
      |           if ~strcmp(s16DerivGainShift_bkup,tmps)
      |             set_param(gcb,'s16DerivGainShift',tmps);
      |           end
      |         end
      |         if isnan(f16LowerLimit)
      |           if ~strcmp(f16LowerLimit_bkup,'0')
      |             set_param(gcb,'f16LowerLimit','0');
      |           end
      |         else
      |           tmps=num2str(f16LowerLimit);
      |           if ~strcmp(f16LowerLimit_bkup,tmps)
      |             set_param(gcb,'f16LowerLimit',tmps);
      |           end
      |         end
      |         if isnan(f16UpperLimit)
      |           if ~strcmp(f16UpperLimit_bkup,'0')
      |             set_param(gcb,'f16UpperLimit','0');
      |           end
      |         else
      |           tmps=num2str(f16UpperLimit);
      |           if ~strcmp(f16UpperLimit_bkup,tmps)
      |             set_param(gcb,'f16UpperLimit',tmps);
      |           end
      |         end
      |       end
      |     end
      |   catch
      |    warning(['Sample time cannot be calculated for the block ' gcb])
      |   end
      | end
      mask DialogControl timeHint Prompt: Note: Implementation parameters cannot be calculated yet because the block's inherited sample time is unknown. Simulink will update the sample time when you run the simulation.
      mask Display:
      | color('black');
      | pos = get_param(gcb, 'Position');
      | width = pos(3) - pos(1);
      | height = pos(4) - pos(2);
      | tX=width/2;
      | tY=height - 25;
      | color('black');
      | text(tX,tY, 'GFLIB_ControllerPIDpAW_F16', 'horizontalAlignment', 'center');
      | if showStates == 2
      |   color('red');
      |   text(tX,tY - 20, ['debugging mode' char(13) char(10) '(limited performance)'], 'horizontalAlignment', 'center');
      | end
  GFLIB_ControllerPIpAW_F16 : Subsystem  StartFcn=|  TreatAsAtomicUnit=on  mask(GFLIB_ControllerPIpAW_F16){showStates=Hide (faster execution), resetStatesEnable=Pre-set according to the first set of inputs after reset, SampleTime=-1, pgain=5, igain=0.5, lowerLimit=-10, upperLimit=9.99969482421875, inscale=10, outscale=10, autoCalcEn=on, f16PropGain=0, f16IntegGain=0, s16PropGainShift=0, s16IntegGainShift=0, f16LowerLimit=0, f16UpperLimit=0, SampleTime_1=NaN}
      | ts=get_param(gcb,'CompiledSampleTime');
      | if iscell(ts)
      |   ts=ts{1};
      |   if iscell(ts)
      |     ts=ts{1};
      |   end
      | end
      | ts=ts(1);
      | set_param(gcb,'SampleTime_1',num2str(ts));
      | p=Simulink.Mask.get(gcb);
      | hintText=p.getDialogControl('timeHint');
      | SampleTime=Simulink.data.evalinGlobal(bdroot,get_param(gcb,'SampleTime'));
      | p=Simulink.Mask.get(gcb);
      | autoCalcEn=get_param(gcb,'autoCalcEn');
      | if strcmp(autoCalcEn,'on')
      |   if SampleTime==-1
      |     hintText.Prompt='Caution: Implementation parameters depend on inherited sample time. Make sure that the sample time of the block''s inputs corresponds to the sampling period in the target application.';
      |   else
      |     hintText.Prompt='Caution: Implementation parameters depend on the sample time. Make sure that the simulation time step corresponds to the sampling period in the target application.';
      |   end
      |   SampleTime=ts;
      |   f16PropGain_bkup=get_param(gcb,'f16PropGain');
      |   f16IntegGain_bkup=get_param(gcb,'f16IntegGain');
      |   s16PropGainShift_bkup=get_param(gcb,'s16PropGainShift');
      |   s16IntegGainShift_bkup=get_param(gcb,'s16IntegGainShift');
      |   f16LowerLimit_bkup=get_param(gcb,'f16LowerLimit');
      |   f16UpperLimit_bkup=get_param(gcb,'f16UpperLimit');
      |   pgain=Simulink.data.evalinGlobal(bdroot,get_param(gcb,'pgain'));
      |   igain=Simulink.data.evalinGlobal(bdroot,get_param(gcb,'igain'));
      |   lowerLimit=Simulink.data.evalinGlobal(bdroot,get_param(gcb,'lowerLimit'));
      |   upperLimit=Simulink.data.evalinGlobal(bdroot,get_param(gcb,'upperLimit'));
      |   inscale=Simulink.data.evalinGlobal(bdroot,get_param(gcb,'inscale'));
      |   outscale=Simulink.data.evalinGlobal(bdroot,get_param(gcb,'outscale'));
      |   if (upperLimit<=lowerLimit)
      |     warning('UpperLimit should be greater than LowerLimit.');
      |   end
      |   if (inscale<=0)
      |     warning('E_max must be positive.');
      |   end
      |   if (outscale<=0)
      |     warning('U_max must be positive.');
      |   end
      |   kpf=pgain*inscale/outscale;
      |   s16PropGainShift=ceil(log2(abs(kpf)));
      |   if s16PropGainShift<-15
      |     s16PropGainShift=-15;
      |   end
      |   if s16PropGainShift>15
      |     s16PropGainShift=15;
      |     warning(['Parameter s16PropGainShift of ' gcb ' exceeds the fixed-point range.']);
      |   end
      |   f16PropGain=round(kpf*2^(-s16PropGainShift)*2^15);
      |   if f16PropGain>2^15-1
      |     f16PropGain=2^15-1;
      |     warning(['Parameter f16PropGain of ' gcb ' exceeds the fixed-point range.']);
      |   end
      |   if f16PropGain<-2^15
      |     f16PropGain=-2^15;
      |     warning(['Parameter f16PropGain of ' gcb ' exceeds the fixed-point range.']);
      |   end
      |   kif=igain*SampleTime*0.5*inscale/outscale;
      |   s16IntegGainShift=ceil(log2(abs(kif)));
      |   if s16IntegGainShift<-15
      |     s16IntegGainShift=-15;
      |   end
      |   if s16IntegGainShift>15
      |     s16IntegGainShift=15;
      |     warning(['Parameter s16IntegGainShift of ' gcb ' exceeds the fixed-point range.']);
      |   end
      |   f16IntegGain=round(kif*2^(-s16IntegGainShift)*2^15);
      |   if f16IntegGain>2^15-1
      |     f16IntegGain=2^15-1;
      |     warning(['Parameter f16IntegGain of ' gcb ' exceeds the fixed-point range.']);
      |   end
      |   if f16IntegGain<-2^15
      |     f16IntegGain=-2^15;
      |     warning(['Parameter f16IntegGain of ' gcb ' exceeds the fixed-point range.']);
      |   end
      |   upperLimitf=upperLimit/outscale;
      |   lowerLimitf=lowerLimit/outscale;
      |   f16UpperLimit=round(upperLimitf*2^15);
      |   if f16UpperLimit>2^15-1
      |     f16UpperLimit=2^15-1;
      |     warning(['Parameter f16UpperLimit of ' gcb ' exceeds the fixed-point range.']);
      |   end
      |   if f16UpperLimit<-2^15
      |     f16UpperLimit=-2^15;
      |     warning(['Parameter f16UpperLimit of ' gcb ' exceeds the fixed-point range.']);
      |   end
      |   f16LowerLimit=round(lowerLimitf*2^15);
      |   if f16LowerLimit>2^15-1
      |     f16LowerLimit=2^15-1;
      |     warning(['Parameter f16LowerLimit of ' gcb ' exceeds the fixed-point range.']);
      |   end
      |   if f16LowerLimit<-2^15
      |     f16LowerLimit=-2^15;
      |     warning(['Parameter f16LowerLimit of ' gcb ' exceeds the fixed-point range.']);
      |   end
      |   if isnan(f16PropGain)
      |     if ~strcmp(f16PropGain_bkup,'0')
      |       set_param(gcb,'f16PropGain','0');
      |     end
      |   else
      |     tmps=num2str(f16PropGain);
      |     if ~strcmp(f16PropGain_bkup,tmps)
      |       set_param(gcb,'f16PropGain',tmps);
      |     end
      |   end
      |   if isnan(f16IntegGain)
      |     if ~strcmp(f16IntegGain_bkup,'0')
      |       set_param(gcb,'f16IntegGain','0');
      |     end
      |   else
      |     tmps=num2str(f16IntegGain);
      |     if ~strcmp(f16IntegGain_bkup,tmps)
      |       set_param(gcb,'f16IntegGain',tmps);
      |     end
      |   end
      |   if isnan(s16PropGainShift)
      |     if ~strcmp(s16PropGainShift_bkup,'0')
      |       set_param(gcb,'s16PropGainShift','0');
      |     end
      |   else
      |     tmps=num2str(s16PropGainShift);
      |     if ~strcmp(s16PropGainShift_bkup,tmps)
      |       set_param(gcb,'s16PropGainShift',tmps);
      |     end
      |   end
      |   if isnan(s16IntegGainShift)
      |     if ~strcmp(s16IntegGainShift_bkup,'0')
      |       set_param(gcb,'s16IntegGainShift','0');
      |     end
      |   else
      |     tmps=num2str(s16IntegGainShift);
      |     if ~strcmp(s16IntegGainShift_bkup,tmps)
      |       set_param(gcb,'s16IntegGainShift',tmps);
      |     end
      |   end
      |   if isnan(f16LowerLimit)
      |     if ~strcmp(f16LowerLimit_bkup,'0')
      |       set_param(gcb,'f16LowerLimit','0');
      |     end
      |   else
      |     tmps=num2str(f16LowerLimit);
      |     if ~strcmp(f16LowerLimit_bkup,tmps)
      |       set_param(gcb,'f16LowerLimit',tmps);
      |     end
      |   end
      |   if isnan(f16UpperLimit)
      |     if ~strcmp(f16UpperLimit_bkup,'0')
      |       set_param(gcb,'f16UpperLimit','0');
      |     end
      |   else
      |     tmps=num2str(f16UpperLimit);
      |     if ~strcmp(f16UpperLimit_bkup,tmps)
      |       set_param(gcb,'f16UpperLimit',tmps);
      |     end
      |   end
      | end
